simulink model "ElevatorPlant_basic"  (R2015b)
settings: Solver=FixedStepDiscrete  SolverMode=SingleTasking  StartTime=0.0  StopTime=10.0  RelTol=1e-3
(part 2 of 3)

== stateflow chart ElevatorPlant_basic/Elevator Plant ==
  state Init_procedure
    state BLK_Init
      %BLK(LPS0)
      %BLK(LPD1)
      %BLK(LPS1)
      %BLK(LPD2)
      %BLK(LPS2)
      %BLK(LPD3)
    state Replacing
      en:
      SCENDI=true;
    state Closing_all_doors
      state Closing0
        state Timer_close
          state Set_tmr
            en: Q_cl=true;
          state Set
            en:PT_cl=5;
            IN_cl=true;
          state Counting
            en:ET_cl = ET_cl + 1;
            Q_cl=false;
          (junction 9948) -> Init_procedure.Closing_all_doors.Closing0.Timer_close.Set_tmr [order 1] : [ET_cl==PT_cl]
          Init_procedure.Closing_all_doors.Closing0.Timer_close.Set_tmr -> (junction 9949)
          (default) -> Init_procedure.Closing_all_doors.Closing0.Timer_close.Set
          Init_procedure.Closing_all_doors.Closing0.Timer_close.Counting -> (junction 9948)
          (junction 9948) -> (junction 9949) [order 2]
          Init_procedure.Closing_all_doors.Closing0.Timer_close.Set -> (junction 9950)
          (junction 9950) -> Init_procedure.Closing_all_doors.Closing0.Timer_close.Counting [order 1] : [ET_cl<PT_cl]
          (junction 9950) -> (junction 9949) [order 2]
        state BUTT_Temp
          state Butt_temp0
            en: BUT_TEMP = 0;
            FLAG_BT=true;
            LPC0=true;
          state Butt_temp1
            en: BUT_TEMP = 1;
            FLAG_BT=true;
            LPC1=true;
          state Butt_temp2
            en: BUT_TEMP = 2;
            FLAG_BT=true;
            LPC2=true;
          state Butt_temp3
            en: BUT_TEMP = 3;
            FLAG_BT=true;
            LPC3=true;
          (default) -> (junction 13774)
          (junction 13774) -> (junction 13496) [order 1] : [not(FLAG_BT)]
          (junction 13496) -> Init_procedure.Closing_all_doors.Closing0.BUTT_Temp.Butt_temp0 [order 1] : [P0]
          Init_procedure.Closing_all_doors.Closing0.BUTT_Temp.Butt_temp0 -> (junction 13782)
          (junction 13774) -> (junction 13776) [order 2]
          (junction 13496) -> (junction 13769) [order 2]
          (junction 13782) -> (junction 13783)
          (junction 13769) -> Init_procedure.Closing_all_doors.Closing0.BUTT_Temp.Butt_temp1 [order 1] : [P1]
          Init_procedure.Closing_all_doors.Closing0.BUTT_Temp.Butt_temp1 -> (junction 13783)
          (junction 13769) -> (junction 13768) [order 2]
          (junction 13783) -> (junction 13784)
          (junction 13768) -> Init_procedure.Closing_all_doors.Closing0.BUTT_Temp.Butt_temp2 [order 1] : [P2]
          Init_procedure.Closing_all_doors.Closing0.BUTT_Temp.Butt_temp2 -> (junction 13784)
          (junction 13768) -> (junction 13771) [order 2]
          (junction 13784) -> (junction 13785)
          (junction 13771) -> Init_procedure.Closing_all_doors.Closing0.BUTT_Temp.Butt_temp3 [order 1] : [P3]
          Init_procedure.Closing_all_doors.Closing0.BUTT_Temp.Butt_temp3 -> (junction 13785)
          (junction 13771) -> (junction 13779) [order 2]
          (junction 13785) -> (junction 13786)
          (junction 13776) -> (junction 13779)
          (junction 13779) -> (junction 13786)
        state Closing
          en: CP0=Q_cl;
        state Stop_Closing
          en: CP0=false;
          LPS0=false;
          LPS1=false;
          LPD1=false;
          LPS2=false;
          LPD2=false;
          LPD3=false;
          FLAG_OD=false;
          OBS=false;
          ET_cl=0;
          IN_cl=false;
        state Flag_position
          en:FLAG=2;
          FLAG_BT=false;
          BUTTON=BUT_TEMP;
        state Closing1
          en:CP0=true;
        state Flag_floor
          en: FLAG=1;
        state Stop_Closing1
          en:CP0=false;
        Init_procedure.Closing_all_doors.Closing0.Closing -> Init_procedure.Closing_all_doors.Closing0.BUTT_Temp
        (default) -> (junction 9915)
        (junction 9915) -> Init_procedure.Closing_all_doors.Closing0.Timer_close [order 1] : [not(FLAG==0) && not(FLAG==4)]
        Init_procedure.Closing_all_doors.Closing0.Timer_close -> (junction 9914)
        (junction 9914) -> Init_procedure.Closing_all_doors.Closing0.Closing [order 1] : [not(PC0)]
        Init_procedure.Closing_all_doors.Closing0.BUTT_Temp -> (junction 13760)
        (junction 9915) -> (junction 9917) [order 2]
        (junction 9914) -> Init_procedure.Closing_all_doors.Closing0.Stop_Closing [order 2]
        (junction 13760) -> (junction 13757)
        Init_procedure.Closing_all_doors.Closing0.Stop_Closing -> (junction 9916)
        (junction 9916) -> Init_procedure.Closing_all_doors.Closing0.Flag_position [order 1] : [FLAG_BT]
        (junction 9916) -> Init_procedure.Closing_all_doors.Closing0.Flag_floor [order 2]
        Init_procedure.Closing_all_doors.Closing0.Flag_position -> (junction 13754)
        (junction 9917) -> Init_procedure.Closing_all_doors.Closing0.Closing1 [order 1] : [not(PC0)]
        Init_procedure.Closing_all_doors.Closing0.Closing1 -> (junction 13749)
        (junction 9917) -> Init_procedure.Closing_all_doors.Closing0.Stop_Closing1 [order 2]
        (junction 13749) -> (junction 13751)
        Init_procedure.Closing_all_doors.Closing0.Flag_floor -> (junction 13754)
        (junction 13754) -> (junction 13757)
        (junction 13757) -> (junction 13765)
        Init_procedure.Closing_all_doors.Closing0.Stop_Closing1 -> (junction 13751)
        (junction 13751) -> (junction 13765)
      state Closing1
        state BUTT_Temp
          state Butt_temp0
            en: BUT_TEMP = 0;
            FLAG_BT=true;
            LPC0=true;
          state Butt_temp1
            en: BUT_TEMP = 1;
            FLAG_BT=true;
            LPC1=true;
          state Butt_temp2
            en: BUT_TEMP = 2;
            FLAG_BT=true;
            LPC2=true;
          state Butt_temp3
            en: BUT_TEMP = 3;
            FLAG_BT=true;
            LPC3=true;
          (default) -> (junction 14037)
          (junction 14037) -> (junction 14038) [order 1] : [not(FLAG_BT)]
          (junction 14038) -> Init_procedure.Closing_all_doors.Closing1.BUTT_Temp.Butt_temp0 [order 1] : [P0]
          Init_procedure.Closing_all_doors.Closing1.BUTT_Temp.Butt_temp0 -> (junction 14039)
          (junction 14037) -> (junction 14046) [order 2]
          (junction 14038) -> (junction 14041) [order 2]
          (junction 14039) -> (junction 14040)
          (junction 14041) -> Init_procedure.Closing_all_doors.Closing1.BUTT_Temp.Butt_temp1 [order 1] : [P1]
          Init_procedure.Closing_all_doors.Closing1.BUTT_Temp.Butt_temp1 -> (junction 14040)
          (junction 14041) -> (junction 14042) [order 2]
          (junction 14040) -> (junction 14043)
          (junction 14042) -> Init_procedure.Closing_all_doors.Closing1.BUTT_Temp.Butt_temp2 [order 1] : [P2]
          Init_procedure.Closing_all_doors.Closing1.BUTT_Temp.Butt_temp2 -> (junction 14043)
          (junction 14042) -> (junction 14044) [order 2]
          (junction 14043) -> (junction 14045)
          (junction 14044) -> Init_procedure.Closing_all_doors.Closing1.BUTT_Temp.Butt_temp3 [order 1] : [P3]
          Init_procedure.Closing_all_doors.Closing1.BUTT_Temp.Butt_temp3 -> (junction 14045)
          (junction 14044) -> (junction 14047) [order 2]
          (junction 14045) -> (junction 14048)
          (junction 14046) -> (junction 14047)
          (junction 14047) -> (junction 14048)
        state Timer_close
          state Set_tmr
            en: Q_cl=true;
          state Set
            en:PT_cl=5;
            IN_cl=true;
          state Counting
            en:ET_cl = ET_cl + 1;
            Q_cl=false;
          (junction 14022) -> Init_procedure.Closing_all_doors.Closing1.Timer_close.Set_tmr [order 1] : [ET_cl==PT_cl]
          Init_procedure.Closing_all_doors.Closing1.Timer_close.Set_tmr -> (junction 14023)
          (default) -> Init_procedure.Closing_all_doors.Closing1.Timer_close.Set
          Init_procedure.Closing_all_doors.Closing1.Timer_close.Counting -> (junction 14022)
          (junction 14022) -> (junction 14023) [order 2]
          Init_procedure.Closing_all_doors.Closing1.Timer_close.Set -> (junction 14024)
          (junction 14024) -> Init_procedure.Closing_all_doors.Closing1.Timer_close.Counting [order 1] : [ET_cl<PT_cl]
          (junction 14024) -> (junction 14023) [order 2]
        state Closing
          en: CP1=Q_cl;
        state Stop_Closing
          en: CP1=false;
          LPS0=false;
          LPS1=false;
          LPD1=false;
          LPS2=false;
          LPD2=false;
          LPD3=false;
          FLAG_OD=false;
          OBS=false;
          ET_cl=0;
          IN_cl=false;
        state Flag_position
          en:FLAG=2;
          FLAG_BT=false;
          BUTTON=BUT_TEMP;
        state Closing1
          en:CP1=true;
        state Flag_floor
          en: FLAG=1;
        state Stop_Closing1
          en:CP1=false;
        Init_procedure.Closing_all_doors.Closing1.Closing -> Init_procedure.Closing_all_doors.Closing1.BUTT_Temp
        (default) -> (junction 13989)
        (junction 13989) -> Init_procedure.Closing_all_doors.Closing1.Timer_close [order 1] : [not(FLAG==0) && not(FLAG==4)]
        Init_procedure.Closing_all_doors.Closing1.Timer_close -> (junction 13990)
        (junction 13990) -> Init_procedure.Closing_all_doors.Closing1.Closing [order 1] : [not(PC1)]
        Init_procedure.Closing_all_doors.Closing1.BUTT_Temp -> (junction 13991)
        (junction 13989) -> (junction 13993) [order 2]
        (junction 13990) -> Init_procedure.Closing_all_doors.Closing1.Stop_Closing [order 2]
        (junction 13991) -> (junction 13995)
        Init_procedure.Closing_all_doors.Closing1.Stop_Closing -> (junction 13992)
        (junction 13992) -> Init_procedure.Closing_all_doors.Closing1.Flag_position [order 1] : [FLAG_BT]
        (junction 13992) -> Init_procedure.Closing_all_doors.Closing1.Flag_floor [order 2]
        Init_procedure.Closing_all_doors.Closing1.Flag_position -> (junction 13996)
        (junction 13993) -> Init_procedure.Closing_all_doors.Closing1.Closing1 [order 1] : [not(PC1)]
        Init_procedure.Closing_all_doors.Closing1.Closing1 -> (junction 13994)
        (junction 13993) -> Init_procedure.Closing_all_doors.Closing1.Stop_Closing1 [order 2]
        (junction 13994) -> (junction 13997)
        Init_procedure.Closing_all_doors.Closing1.Flag_floor -> (junction 13996)
        (junction 13996) -> (junction 13995)
        (junction 13995) -> (junction 13998)
        Init_procedure.Closing_all_doors.Closing1.Stop_Closing1 -> (junction 13997)
        (junction 13997) -> (junction 13998)
      state Closing2
        state Timer_close
          state Set_tmr
            en: Q_cl=true;
          state Set
            en:PT_cl=5;
            IN_cl=true;
          state Counting
            en:ET_cl = ET_cl + 1;
            Q_cl=false;
          (junction 14114) -> Init_procedure.Closing_all_doors.Closing2.Timer_close.Set_tmr [order 1] : [ET_cl==PT_cl]
          Init_procedure.Closing_all_doors.Closing2.Timer_close.Set_tmr -> (junction 14115)
          (default) -> Init_procedure.Closing_all_doors.Closing2.Timer_close.Set
          Init_procedure.Closing_all_doors.Closing2.Timer_close.Counting -> (junction 14114)
          (junction 14114) -> (junction 14115) [order 2]
          Init_procedure.Closing_all_doors.Closing2.Timer_close.Set -> (junction 14116)
          (junction 14116) -> Init_procedure.Closing_all_doors.Closing2.Timer_close.Counting [order 1] : [ET_cl<PT_cl]
          (junction 14116) -> (junction 14115) [order 2]
        state BUTT_Temp
          state Butt_temp0
            en: BUT_TEMP = 0;
            FLAG_BT=true;
            LPC0=true;
          state Butt_temp1
            en: BUT_TEMP = 1;
            FLAG_BT=true;
            LPC1=true;
          state Butt_temp2
            en: BUT_TEMP = 2;
            FLAG_BT=true;
            LPC2=true;
          state Butt_temp3
            en: BUT_TEMP = 3;
            FLAG_BT=true;
            LPC3=true;
          (default) -> (junction 14129)
          (junction 14129) -> (junction 14130) [order 1] : [not(FLAG_BT)]
          (junction 14130) -> Init_procedure.Closing_all_doors.Closing2.BUTT_Temp.Butt_temp0 [order 1] : [P0]
          Init_procedure.Closing_all_doors.Closing2.BUTT_Temp.Butt_temp0 -> (junction 14131)
          (junction 14129) -> (junction 14138) [order 2]
          (junction 14130) -> (junction 14133) [order 2]
          (junction 14131) -> (junction 14132)
          (junction 14133) -> Init_procedure.Closing_all_doors.Closing2.BUTT_Temp.Butt_temp1 [order 1] : [P1]
          Init_procedure.Closing_all_doors.Closing2.BUTT_Temp.Butt_temp1 -> (junction 14132)
          (junction 14133) -> (junction 14134) [order 2]
          (junction 14132) -> (junction 14135)
          (junction 14134) -> Init_procedure.Closing_all_doors.Closing2.BUTT_Temp.Butt_temp2 [order 1] : [P2]
          Init_procedure.Closing_all_doors.Closing2.BUTT_Temp.Butt_temp2 -> (junction 14135)
          (junction 14134) -> (junction 14136) [order 2]
          (junction 14135) -> (junction 14137)
          (junction 14136) -> Init_procedure.Closing_all_doors.Closing2.BUTT_Temp.Butt_temp3 [order 1] : [P3]
          Init_procedure.Closing_all_doors.Closing2.BUTT_Temp.Butt_temp3 -> (junction 14137)
          (junction 14136) -> (junction 14139) [order 2]
          (junction 14137) -> (junction 14140)
          (junction 14138) -> (junction 14139)
          (junction 14139) -> (junction 14140)
        state Closing
          en: CP2=Q_cl;
        state Stop_Closing
          en: CP2=false;
          LPS0=false;
          LPS1=false;
          LPD1=false;
          LPS2=false;
          LPD2=false;
          LPD3=false;
          FLAG_OD=false;
          OBS=false;
          ET_cl=0;
          IN_cl=false;
        state Flag_position
          en:FLAG=2;
          FLAG_BT=false;
          BUTTON=BUT_TEMP;
        state Closing1
          en:CP2=true;
        state Flag_floor
          en: FLAG=1;
        state Stop_Closing1
          en:CP2=false;
        Init_procedure.Closing_all_doors.Closing2.Closing -> Init_procedure.Closing_all_doors.Closing2.BUTT_Temp
        (default) -> (junction 14081)
        (junction 14081) -> Init_procedure.Closing_all_doors.Closing2.Timer_close [order 1] : [not(FLAG==0) && not(FLAG==4)]
        Init_procedure.Closing_all_doors.Closing2.Timer_close -> (junction 14082)
        (junction 14082) -> Init_procedure.Closing_all_doors.Closing2.Closing [order 1] : [not(PC2)]
        Init_procedure.Closing_all_doors.Closing2.BUTT_Temp -> (junction 14083)
        (junction 14081) -> (junction 14085) [order 2]
        (junction 14082) -> Init_procedure.Closing_all_doors.Closing2.Stop_Closing [order 2]
        (junction 14083) -> (junction 14087)
        Init_procedure.Closing_all_doors.Closing2.Stop_Closing -> (junction 14084)
        (junction 14084) -> Init_procedure.Closing_all_doors.Closing2.Flag_position [order 1] : [FLAG_BT]
        (junction 14084) -> Init_procedure.Closing_all_doors.Closing2.Flag_floor [order 2]
        Init_procedure.Closing_all_doors.Closing2.Flag_position -> (junction 14088)
        (junction 14085) -> Init_procedure.Closing_all_doors.Closing2.Closing1 [order 1] : [not(PC2)]
        Init_procedure.Closing_all_doors.Closing2.Closing1 -> (junction 14086)
        (junction 14085) -> Init_procedure.Closing_all_doors.Closing2.Stop_Closing1 [order 2]
        (junction 14086) -> (junction 14089)
        Init_procedure.Closing_all_doors.Closing2.Flag_floor -> (junction 14088)
        (junction 14088) -> (junction 14087)
        (junction 14087) -> (junction 14090)
        Init_procedure.Closing_all_doors.Closing2.Stop_Closing1 -> (junction 14089)
        (junction 14089) -> (junction 14090)
      state Closing3
        state Timer_close
          state Set_tmr
            en: Q_cl=true;
          state Set
            en:PT_cl=5;
            IN_cl=true;
          state Counting
            en:ET_cl = ET_cl + 1;
            Q_cl=false;
          (junction 14206) -> Init_procedure.Closing_all_doors.Closing3.Timer_close.Set_tmr [order 1] : [ET_cl==PT_cl]
          Init_procedure.Closing_all_doors.Closing3.Timer_close.Set_tmr -> (junction 14207)
          (default) -> Init_procedure.Closing_all_doors.Closing3.Timer_close.Set
          Init_procedure.Closing_all_doors.Closing3.Timer_close.Counting -> (junction 14206)
          (junction 14206) -> (junction 14207) [order 2]
          Init_procedure.Closing_all_doors.Closing3.Timer_close.Set -> (junction 14208)
          (junction 14208) -> Init_procedure.Closing_all_doors.Closing3.Timer_close.Counting [order 1] : [ET_cl<PT_cl]
          (junction 14208) -> (junction 14207) [order 2]
        state BUTT_Temp
          state Butt_temp0
            en: BUT_TEMP = 0;
            FLAG_BT=true;
            LPC0=true;
          state Butt_temp1
            en: BUT_TEMP = 1;
            FLAG_BT=true;
            LPC1=true;
          state Butt_temp2
            en: BUT_TEMP = 2;
            FLAG_BT=true;
            LPC2=true;
          state Butt_temp3
            en: BUT_TEMP = 3;
            FLAG_BT=true;
            LPC3=true;
          (default) -> (junction 14221)
          (junction 14221) -> (junction 14222) [order 1] : [not(FLAG_BT)]
          (junction 14222) -> Init_procedure.Closing_all_doors.Closing3.BUTT_Temp.Butt_temp0 [order 1] : [P0]
          Init_procedure.Closing_all_doors.Closing3.BUTT_Temp.Butt_temp0 -> (junction 14223)
          (junction 14221) -> (junction 14230) [order 2]
          (junction 14222) -> (junction 14225) [order 2]
          (junction 14223) -> (junction 14224)
          (junction 14225) -> Init_procedure.Closing_all_doors.Closing3.BUTT_Temp.Butt_temp1 [order 1] : [P1]
          Init_procedure.Closing_all_doors.Closing3.BUTT_Temp.Butt_temp1 -> (junction 14224)
          (junction 14225) -> (junction 14226) [order 2]
          (junction 14224) -> (junction 14227)
          (junction 14226) -> Init_procedure.Closing_all_doors.Closing3.BUTT_Temp.Butt_temp2 [order 1] : [P2]
          Init_procedure.Closing_all_doors.Closing3.BUTT_Temp.Butt_temp2 -> (junction 14227)
          (junction 14226) -> (junction 14228) [order 2]
          (junction 14227) -> (junction 14229)
          (junction 14228) -> Init_procedure.Closing_all_doors.Closing3.BUTT_Temp.Butt_temp3 [order 1] : [P3]
          Init_procedure.Closing_all_doors.Closing3.BUTT_Temp.Butt_temp3 -> (junction 14229)
          (junction 14228) -> (junction 14231) [order 2]
          (junction 14229) -> (junction 14232)
          (junction 14230) -> (junction 14231)
          (junction 14231) -> (junction 14232)
        state Closing
          en: CP3=Q_cl;
        state Stop_Closing
          en: CP3=false;
          LPS0=false;
          LPS1=false;
          LPD1=false;
          LPS2=false;
          LPD2=false;
          LPD3=false;
          FLAG_OD=false;
          OBS=false;
          ET_cl=0;
          IN_cl=false;
        state Flag_position
          en:FLAG=2;
          FLAG_BT=false;
          BUTTON=BUT_TEMP;
        state Closing1
          en:CP3=true;
        state Flag_floor
          en: FLAG=1;
        state Stop_Closing1
          en:CP3=false;
        Init_procedure.Closing_all_doors.Closing3.Closing -> Init_procedure.Closing_all_doors.Closing3.BUTT_Temp
        (default) -> (junction 14173)
        (junction 14173) -> Init_procedure.Closing_all_doors.Closing3.Timer_close [order 1] : [not(FLAG==0) && not(FLAG==4)]
        Init_procedure.Closing_all_doors.Closing3.Timer_close -> (junction 14174)
        (junction 14174) -> Init_procedure.Closing_all_doors.Closing3.Closing [order 1] : [not(PC3)]
        Init_procedure.Closing_all_doors.Closing3.BUTT_Temp -> (junction 14175)
        (junction 14173) -> (junction 14177) [order 2]
        (junction 14174) -> Init_procedure.Closing_all_doors.Closing3.Stop_Closing [order 2]
        (junction 14175) -> (junction 14179)
        Init_procedure.Closing_all_doors.Closing3.Stop_Closing -> (junction 14176)
        (junction 14176) -> Init_procedure.Closing_all_doors.Closing3.Flag_position [order 1] : [FLAG_BT]
        (junction 14176) -> Init_procedure.Closing_all_doors.Closing3.Flag_floor [order 2]
        Init_procedure.Closing_all_doors.Closing3.Flag_position -> (junction 14180)
        (junction 14177) -> Init_procedure.Closing_all_doors.Closing3.Closing1 [order 1] : [not(PC3)]
        Init_procedure.Closing_all_doors.Closing3.Closing1 -> (junction 14178)
        (junction 14177) -> Init_procedure.Closing_all_doors.Closing3.Stop_Closing1 [order 2]
        (junction 14178) -> (junction 14181)
        Init_procedure.Closing_all_doors.Closing3.Flag_floor -> (junction 14180)
        (junction 14180) -> (junction 14179)
        (junction 14179) -> (junction 14182)
        Init_procedure.Closing_all_doors.Closing3.Stop_Closing1 -> (junction 14181)
        (junction 14181) -> (junction 14182)
      (default) -> Init_procedure.Closing_all_doors.Closing0
      Init_procedure.Closing_all_doors.Closing1 -> Init_procedure.Closing_all_doors.Closing2
      Init_procedure.Closing_all_doors.Closing0 -> Init_procedure.Closing_all_doors.Closing1
      Init_procedure.Closing_all_doors.Closing2 -> Init_procedure.Closing_all_doors.Closing3
    state Replaced
      en:
      SCENDI=false;
    state End_init
      en:
      LPS0=false;LPS1=false;
      LPS2=false;LPD2=false;
      LPD3=false;LPD1=false;
      FLAG=1;
    Init_procedure.Replacing -> (junction 13744)
    BLK_Init -> Closing_all_doors
    Closing_all_doors -> (junction 4531)
    (junction 4531) -> Init_procedure.Replacing [order 1] : [not(RPC0) && not(RPC1) && not(RPC2) && not(RPC3)]
    (default) -> BLK_Init
    (junction 13744) -> (junction 13732)
    (junction 4531) -> Init_procedure.Replaced [order 2]
    Init_procedure.Replaced -> (junction 13732)
    (junction 13732) -> (junction 13735)
    (junction 13735) -> (junction 13739) [order 2]
    (junction 13735) -> End_init [order 1] : [(RPC0 ||RPC1 ||RPC2 ||RPC3) && (PC0 && PC1 && PC2 && PC3)]
    (junction 13739) -> (junction 13741)
    End_init -> (junction 13737)
    (junction 13737) -> (junction 13741)
  state Blackout
    state OFF
      en:	FLAG_BO=true;
      AP0=false;
      AP1=false;
      AP2=false;
      AP3=false;
      CP0=false;
      CP1=false;
      CP2=false;
      CP3=false;
      SALI=false;
      SCENDI=false;
      LL=false;
      LPC0=false;
      LPC1=false;
      LPC2=false;
      LPC3=false;
      LPS0=false;
      LPS1=false;
      LPD1=false;
      LPS2=false;
      LPD2=false;
      LPD3=false;
      FLAG=5;
      IN_LL=false; ET_LL=0;
    state Start_recovery
      en:
      FLAG_REC=true;
      FLAG=4;
    state ON
      en:
      LL=true;
    state Recovery_finished
    OFF -> (junction 13581)
    (default) -> (junction 4492)
    (junction 4492) -> OFF [order 1] : [BO && not(FLAG_BO) && not(RECOVERY)]
    (junction 4492) -> (junction 13599) [order 2]
    (junction 13581) -> Start_recovery [order 1] : [RECOVERY]
    Start_recovery -> (junction 13584)
    (junction 13599) -> ON [order 1] : [not(BO) && not(RECOVERY)]
    ON -> (junction 13581)
    (junction 13581) -> Recovery_finished [order 2]
    Recovery_finished -> (junction 13584)
    (junction 13599) -> (junction 13728) [order 2]
    (junction 13726) -> (junction 13581)
    (junction 13728) -> (junction 13726)
  state Fire_detection
    state Firing
      en:FLAG=4;
      FLAG_EMG=true;
      SALI=false;
    state NOT_fire
    (default) -> (junction 13568)
    (junction 13568) -> Firing [order 1] : [FIRE]
    Firing -> (junction 13579)
    (junction 13568) -> NOT_fire [order 2]
    NOT_fire -> (junction 13579)
  state Floor_detection
    state F0
      en:
      FLOOR=0;
      LPC0=true;
    state No_floor
    state NOT_F0
      en:
      LPC0=false;
    state F1
      en:
      FLOOR=1;
      LPC1=true;
    state NOT_F1
      en:
      LPC1=false;
    state F2
      en:
      FLOOR=2;
      LPC2=true;
    state NOT_F2
      en:
      LPC2=false;
    state F3
      en:
      FLOOR=3;
      LPC3=true;
    state F4
      en:
      LPC3=false;
    (junction 4501) -> F0 [order 1] : [RPC0]
    Floor_detection.No_floor -> (junction 4501)
    F0 -> (junction 13681)
    (default) -> Floor_detection.No_floor
    (junction 4501) -> (junction 13667) [order 2]
    (junction 13667) -> NOT_F0 [order 1] : [not(BUT_TEMP==0)]
    NOT_F0 -> (junction 13681)
    (junction 13667) -> (junction 13684) [order 2]
    (junction 13681) -> (junction 13707)
    (junction 13707) -> (junction 13684)
    (junction 13684) -> (junction 4502)
    (junction 4502) -> F1 [order 1] : [RPC1]
    (junction 4502) -> (junction 13669) [order 2]
    F1 -> (junction 13688)
    (junction 13669) -> NOT_F1 [order 1] : [not(BUT_TEMP==1)]
    (junction 13669) -> (junction 13691) [order 2]
    NOT_F1 -> (junction 13688)
    (junction 13688) -> (junction 13705)
    (junction 13705) -> (junction 13691)
    (junction 13691) -> (junction 4503)
    (junction 4503) -> F2 [order 1] : [RPC2]
    F2 -> (junction 13709)
    (junction 4503) -> (junction 13671) [order 2]
    (junction 13671) -> NOT_F2 [order 1] : [not(BUT_TEMP==2)]
    NOT_F2 -> (junction 13709)
    (junction 13671) -> (junction 13695) [order 2]
    (junction 13709) -> (junction 13702)
    (junction 13702) -> (junction 13695)
    (junction 13695) -> (junction 4504)
    F3 -> (junction 13710)
    (junction 4504) -> F3 [order 1] : [RPC3]
    (junction 4504) -> (junction 13673) [order 2]
    (junction 13673) -> F4 [order 1] : [not(BUT_TEMP==3)]
    F4 -> (junction 13710)
    (junction 13673) -> (junction 13715) [order 2]
    (junction 13710) -> (junction 13713)
    (junction 13715) -> (junction 13713)
  state Button_detection
    state BUTTON_0
      en:
      BUTTON=0;
      FLAG=2;
      IN_LL=false; ET_LL=0;
    state No_button
    state Supply_OFF
      en:
      LL=not(Q_LL);
    state Timer_LL
      state Set_tmr
        en:
        Q_LL=true;
      state Counting
        en:
        ET_LL = ET_LL + 1;
        Q_LL=false;
      state Set
        en:
        IN_LL=true;
        PT_LL=10;
      (junction 4546) -> Button_detection.Timer_LL.Set_tmr [order 1] : [ET_LL==PT_LL]
      Button_detection.Timer_LL.Set_tmr -> (junction 4547)
      Button_detection.Timer_LL.Counting -> (junction 4546)
      (junction 4546) -> (junction 4547) [order 2]
      (default) -> Button_detection.Timer_LL.Set
      Button_detection.Timer_LL.Set -> (junction 4545)
      (junction 4545) -> Button_detection.Timer_LL.Counting [order 1] : [ET_LL<PT_LL]
      (junction 4545) -> (junction 4547) [order 2]
    state BUTTON_1
      en:
      BUTTON=1;
      FLAG=2;
      IN_LL=false; ET_LL=0;
    state BUTTON_2
      en:
      BUTTON=2;
      FLAG=2;
      IN_LL=false; ET_LL=0;
    state BUTTON_3
      en:
      BUTTON=3;
      FLAG=2;
      IN_LL=false; ET_LL=0;
    state STOP
      en:
      IN_LL=false; ET_LL=0;
      FLAG=1;
    state Timer_EME
      state Set_tmr
        en:
        Q_EME=true;
      state Counting
        en:
        ET_EME= ET_EME + 1;
        Q_EME=false;
      state Set
        en:
        IN_EME=true;
        PT_EME=3;
      (junction 4593) -> Button_detection.Timer_EME.Set_tmr [order 1] : [ET_EME==PT_EME]
      Button_detection.Timer_EME.Set_tmr -> (junction 4594)
      Button_detection.Timer_EME.Counting -> (junction 4593)
      (junction 4593) -> (junction 4594) [order 2]
      (default) -> Button_detection.Timer_EME.Set
      Button_detection.Timer_EME.Set -> (junction 4595)
      (junction 4595) -> Button_detection.Timer_EME.Counting [order 1] : [ET_EME<PT_EME]
      (junction 4595) -> (junction 4594) [order 2]
    state EME
      en:
      FLAG_EME=true;
      FLAG=4;
    state Remain_here
      en:
      FLAG=1;
    state NOT_STOP
      en:
      IN_EME=false;
      ET_EME=0;
    (default) -> No_button
    (junction 14266) -> Timer_LL [order 1] : [FLAG_STOP]
    Supply_OFF -> (junction 4167)
    (junction 4167) -> BUTTON_0 [order 1] : [P0|| PS0]
    BUTTON_0 -> (junction 14276)
    No_button -> (junction 14266)
    Timer_LL -> Supply_OFF
    (junction 14266) -> (junction 14295) [order 2]
    (junction 4167) -> (junction 14268) [order 2]
    (junction 14276) -> (junction 14277)
    (junction 14268) -> BUTTON_1 [order 1] : [P1|| PS1|| PD1]
    BUTTON_1 -> (junction 14277)
    (junction 14268) -> (junction 14270) [order 2]
    (junction 14277) -> (junction 14278)
    (junction 14270) -> BUTTON_2 [order 1] : [P2 || PS2 || PD2]
    BUTTON_2 -> (junction 14278)
    (junction 14270) -> (junction 14272) [order 2]
    (junction 14278) -> (junction 14279)
    (junction 25236) -> (junction 14291) [order 2]
    (junction 14272) -> BUTTON_3 [order 1] : [P3 || PD3]
    BUTTON_3 -> (junction 14279)
    (junction 14272) -> Remain_here [order 2]
    (junction 14279) -> (junction 14289)
    (junction 4567) -> STOP [order 1] : [STOP]
    STOP -> Timer_EME
    Timer_EME -> (junction 25236)
    (junction 25236) -> EME [order 1] : [Q_EME]
    EME -> (junction 14291)
    NOT_STOP -> (junction 14291)
    (junction 14291) -> (junction 14297)
    Remain_here -> (junction 14289)
    (junction 14289) -> (junction 4567) : {BUT_TEMP=BUTTON}
    (junction 4567) -> NOT_STOP [order 2]
    (junction 14295) -> (junction 14297)
  state Position_control
    state BUSY
      en:LPS0=true;
      LPS1=true;
      LPD1=true;
      LPS2=true;
      LPD2=true;
      LPD3=true;
    state MOVING_UP
      en:SALI=true;
      MOTION=0;
      FLAG_STOP=false;
      %BLK_TARGET()
    state MOVING_DOWN
      en:SCENDI=true;
      MOTION=1;
      FLAG_STOP=false;
      %BLK_TARGET()
    state AFTER_STOP
      state DOWN_STOP
        en: SCENDI=true;
        %BLK_TARGET();
      state NOT_DOWN
        en: FLAG_STOP=false;
      state UP_STOP
        en: SALI=true;
        %BLK_TARGET();
      state NOT_UP
        en: FLAG_STOP=false;
      (default) -> (junction 8506)
      (junction 8506) -> (junction 8505) [order 1] : [MOTION==0]
      (junction 8505) -> DOWN_STOP [order 1] : [not(( RPC0==true && BUTTON==0)||( RPC1==true && BUTTON==1)||( RPC2==true && BUTTON==2)||( RPC3==true && BUTTON==3)||(STOP==true))]
      (junction 8506) -> (junction 8507) [order 2] : [MOTION==1]
      (junction 8505) -> NOT_DOWN [order 2]
      DOWN_STOP -> (junction 14323)
      NOT_DOWN -> (junction 14323)
      (junction 14323) -> (junction 14326)
      (junction 8507) -> UP_STOP [order 1] : [not(( RPC0==true && BUTTON==0)||( RPC1==true && BUTTON==1)||( RPC2==true && BUTTON==2)||( RPC3==true && BUTTON==3)||(STOP==true))]
      (junction 8507) -> NOT_UP [order 2]
      UP_STOP -> (junction 14320)
      NOT_UP -> (junction 14320)
      (junction 14320) -> (junction 14326)
    state FINISH_POSITIONING
      en:FLAG=3;
    state STOP_CONDITION
      en:FLAG=1;
      FLAG_STOP=true;
    (default) -> BUSY
    BUSY -> (junction 8494)
    (junction 8494) -> MOVING_UP [order 1] : [BUTTON>FLOOR && not(STOP)]
    MOVING_UP -> (junction 14309)
    (junction 8494) -> (junction 14302) [order 2]
    (junction 14309) -> (junction 14310)
    (junction 14302) -> MOVING_DOWN [order 1] : [BUTTON<FLOOR && not(STOP)]
    MOVING_DOWN -> (junction 14310)
    (junction 14302) -> (junction 14305) [order 2]
    (junction 14310) -> (junction 14311)
    (junction 14305) -> AFTER_STOP [order 1] : [BUTTON==FLOOR && FLAG_STOP]
    AFTER_STOP -> (junction 14311)
    (junction 14305) -> (junction 25225) [order 2] : {SALI=false;
        | SCENDI=false;
        | LPC0=false;
        | LPC1=false;
        | LPC2=false;
        | LPC3=false;}
    (junction 14311) -> (junction 14317)
    (junction 25225) -> FINISH_POSITIONING [order 1] : [RPC0==true ||RPC1==true ||RPC2==true ||RPC3==true]
    (junction 25225) -> STOP_CONDITION [order 2]
    FINISH_POSITIONING -> (junction 25226)
    (junction 25226) -> (junction 14317)
    STOP_CONDITION -> (junction 25226)
  state OpCl_doors
    state OpCl_0
      state Closing0
        state Timer_close
          state Set_tmr
            en: Q_cl=true;
          state Set
            en:PT_cl=5;
            IN_cl=true;
          state Counting
            en:ET_cl = ET_cl + 1;
            Q_cl=false;
          (junction 14764) -> OpCl_doors.OpCl_0.Closing0.Timer_close.Set_tmr [order 1] : [ET_cl==PT_cl]
          OpCl_doors.OpCl_0.Closing0.Timer_close.Set_tmr -> (junction 14765)
          (default) -> OpCl_doors.OpCl_0.Closing0.Timer_close.Set
          OpCl_doors.OpCl_0.Closing0.Timer_close.Counting -> (junction 14764)
          (junction 14764) -> (junction 14765) [order 2]
          OpCl_doors.OpCl_0.Closing0.Timer_close.Set -> (junction 14766)
          (junction 14766) -> OpCl_doors.OpCl_0.Closing0.Timer_close.Counting [order 1] : [ET_cl<PT_cl]
          (junction 14766) -> (junction 14765) [order 2]
        state BUTT_Temp
          state Butt_temp0
            en: BUT_TEMP = 0;
            FLAG_BT=true;
            LPC0=true;
          state Butt_temp1
            en: BUT_TEMP = 1;
            FLAG_BT=true;
            LPC1=true;
          state Butt_temp2
            en: BUT_TEMP = 2;
            FLAG_BT=true;
            LPC2=true;
          state Butt_temp3
            en: BUT_TEMP = 3;
            FLAG_BT=true;
            LPC3=true;
          (default) -> (junction 14779)
          (junction 14779) -> (junction 14780) [order 1] : [not(FLAG_BT)]
          (junction 14780) -> OpCl_doors.OpCl_0.Closing0.BUTT_Temp.Butt_temp0 [order 1] : [P0]
          OpCl_doors.OpCl_0.Closing0.BUTT_Temp.Butt_temp0 -> (junction 14781)
          (junction 14779) -> (junction 14788) [order 2]
          (junction 14780) -> (junction 14783) [order 2]
          (junction 14781) -> (junction 14782)
          (junction 14783) -> OpCl_doors.OpCl_0.Closing0.BUTT_Temp.Butt_temp1 [order 1] : [P1]
          OpCl_doors.OpCl_0.Closing0.BUTT_Temp.Butt_temp1 -> (junction 14782)
          (junction 14783) -> (junction 14784) [order 2]
          (junction 14782) -> (junction 14785)
          (junction 14784) -> OpCl_doors.OpCl_0.Closing0.BUTT_Temp.Butt_temp2 [order 1] : [P2]
          OpCl_doors.OpCl_0.Closing0.BUTT_Temp.Butt_temp2 -> (junction 14785)
          (junction 14784) -> (junction 14786) [order 2]
          (junction 14785) -> (junction 14787)
          (junction 14786) -> OpCl_doors.OpCl_0.Closing0.BUTT_Temp.Butt_temp3 [order 1] : [P3]
          OpCl_doors.OpCl_0.Closing0.BUTT_Temp.Butt_temp3 -> (junction 14787)
          (junction 14786) -> (junction 14789) [order 2]
          (junction 14787) -> (junction 14790)
          (junction 14788) -> (junction 14789)
          (junction 14789) -> (junction 14790)
        state Closing
          en: CP0=Q_cl;
        state Stop_Closing
          en: CP0=false;
          LPS0=false;
          LPS1=false;
          LPD1=false;
          LPS2=false;
          LPD2=false;
          LPD3=false;
          FLAG_OD=false;
          OBS=false;
          ET_cl=0;
          IN_cl=false;
        state Flag_position
          en:FLAG=2;
          FLAG_BT=false;
          BUTTON=BUT_TEMP;
        state Closing1
          en:CP0=true;
        state Flag_floor
          en: FLAG=1;
        state Stop_Closing1
          en:CP0=false;
        OpCl_doors.OpCl_0.Closing0.Closing -> OpCl_doors.OpCl_0.Closing0.BUTT_Temp
        (default) -> (junction 14731)
        (junction 14731) -> OpCl_doors.OpCl_0.Closing0.Timer_close [order 1] : [not(FLAG==0) && not(FLAG==4)]
        OpCl_doors.OpCl_0.Closing0.Timer_close -> (junction 14732)
        (junction 14732) -> OpCl_doors.OpCl_0.Closing0.Closing [order 1] : [not(PC0)]
        OpCl_doors.OpCl_0.Closing0.BUTT_Temp -> (junction 14733)
        (junction 14731) -> (junction 14735) [order 2]
        (junction 14732) -> OpCl_doors.OpCl_0.Closing0.Stop_Closing [order 2]
        (junction 14733) -> (junction 14737)
        OpCl_doors.OpCl_0.Closing0.Stop_Closing -> (junction 14734)
        (junction 14734) -> OpCl_doors.OpCl_0.Closing0.Flag_position [order 1] : [FLAG_BT]
        (junction 14734) -> OpCl_doors.OpCl_0.Closing0.Flag_floor [order 2]
        OpCl_doors.OpCl_0.Closing0.Flag_position -> (junction 14738)
        (junction 14735) -> OpCl_doors.OpCl_0.Closing0.Closing1 [order 1] : [not(PC0)]
        OpCl_doors.OpCl_0.Closing0.Closing1 -> (junction 14736)
        (junction 14735) -> OpCl_doors.OpCl_0.Closing0.Stop_Closing1 [order 2]
        (junction 14736) -> (junction 14739)
        OpCl_doors.OpCl_0.Closing0.Flag_floor -> (junction 14738)
        (junction 14738) -> (junction 14737)
        (junction 14737) -> (junction 14740)
        OpCl_doors.OpCl_0.Closing0.Stop_Closing1 -> (junction 14739)
        (junction 14739) -> (junction 14740)
      state StopClosing
        en: CP0=false;
        FLAG_OD=false;
      state Opening0
        state Opening
          en:AP0=Q_op;
        state Stop_Opening
          en:AP0=false;
          FLAG_OD=true;
          OBS=true;
          IN_op=false;
          ET_op=0;
        state Timer_open
          state Set_tmr
            en: Q_op=true;
          state Set
            en:PT_op=2;
            IN_op=true;
          state Counting
            en:ET_op = ET_op + 1;
            Q_op=false;
          (junction 15302) -> OpCl_doors.OpCl_0.Opening0.Timer_open.Set_tmr [order 1] : [ET_op==PT_op]
          OpCl_doors.OpCl_0.Opening0.Timer_open.Set_tmr -> (junction 15303)
          (default) -> OpCl_doors.OpCl_0.Opening0.Timer_open.Set
          OpCl_doors.OpCl_0.Opening0.Timer_open.Counting -> (junction 15302)
          (junction 15302) -> (junction 15303) [order 2]
          OpCl_doors.OpCl_0.Opening0.Timer_open.Set -> (junction 15304)
          (junction 15304) -> OpCl_doors.OpCl_0.Opening0.Timer_open.Counting [order 1] : [ET_op<PT_op]
          (junction 15304) -> (junction 15303) [order 2]
        state BUTT_Temp
          state Butt_temp0
            en: BUT_TEMP = 0;
            FLAG_BT=true;
            LPC0=true;
          state Butt_temp1
            en: BUT_TEMP = 1;
            FLAG_BT=true;
            LPC1=true;
          state Butt_temp2
            en: BUT_TEMP = 2;
            FLAG_BT=true;
            LPC2=true;
          state Butt_temp3
            en: BUT_TEMP = 3;
            FLAG_BT=true;
            LPC3=true;
          (default) -> (junction 20090)
          (junction 20090) -> (junction 20091) [order 1] : [not(FLAG_BT)]
          (junction 20091) -> OpCl_doors.OpCl_0.Opening0.BUTT_Temp.Butt_temp0 [order 1] : [P0]
          OpCl_doors.OpCl_0.Opening0.BUTT_Temp.Butt_temp0 -> (junction 20092)
          (junction 20091) -> (junction 20094) [order 2]
          (junction 20092) -> (junction 20093)
          (junction 20090) -> (junction 20101) [order 2]
          OpCl_doors.OpCl_0.Opening0.BUTT_Temp.Butt_temp1 -> (junction 20093)
          (junction 20094) -> OpCl_doors.OpCl_0.Opening0.BUTT_Temp.Butt_temp1 [order 1] : [P1]
          (junction 20093) -> (junction 20096)
          (junction 20094) -> (junction 20095) [order 2]
          (junction 20095) -> OpCl_doors.OpCl_0.Opening0.BUTT_Temp.Butt_temp2 [order 1] : [P2]
          OpCl_doors.OpCl_0.Opening0.BUTT_Temp.Butt_temp2 -> (junction 20096)
          (junction 20095) -> (junction 20097) [order 2]
          (junction 20096) -> (junction 20098)
          (junction 20097) -> OpCl_doors.OpCl_0.Opening0.BUTT_Temp.Butt_temp3 [order 1] : [P3]
          OpCl_doors.OpCl_0.Opening0.BUTT_Temp.Butt_temp3 -> (junction 20098)
          (junction 20098) -> (junction 20100)
          (junction 20097) -> (junction 20099) [order 2]
          (junction 20100) -> (junction 20099)
          (junction 20099) -> (junction 20102)
          (junction 20101) -> (junction 20102)
        state People_IN
          state Check_People_IN
            en:
            COUNTER_IN=false;
          state Ready_IN
            en:
            IN_DEL_IN=false;
            ET_DEL_IN=0;
          state People_KID_IN
            en:
            WEIGHT=WEIGHT+30;
            KIDS=KIDS+1;
          state DELAY_IN
            state Set_tmr
              en:
              Q_DEL_IN=true;
            state Counting
              en:
              ET_DEL_IN = ET_DEL_IN + 1;
              Q_DEL_IN=false;
            state Set
              en:
              IN_DEL_IN=true;
              PT_DEL_IN=0.05;
            (junction 15383) -> OpCl_doors.OpCl_0.Opening0.People_IN.DELAY_IN.Set_tmr [order 1] : [ET_DEL_IN==PT_DEL_IN]
            OpCl_doors.OpCl_0.Opening0.People_IN.DELAY_IN.Set_tmr -> (junction 15384)
            OpCl_doors.OpCl_0.Opening0.People_IN.DELAY_IN.Counting -> (junction 15383)
            (junction 15383) -> (junction 15384) [order 2]
            (default) -> OpCl_doors.OpCl_0.Opening0.People_IN.DELAY_IN.Set
            OpCl_doors.OpCl_0.Opening0.People_IN.DELAY_IN.Set -> (junction 15385)
            (junction 15385) -> OpCl_doors.OpCl_0.Opening0.People_IN.DELAY_IN.Counting [order 1] : [ET_DEL_IN<PT_DEL_IN]
            (junction 15385) -> (junction 15384) [order 2]
          state People_WOMAN_IN
            en:
            WEIGHT=WEIGHT+55;
            WOMEN=WOMEN+1;
          state People_MAN_IN
            en:
            WEIGHT=WEIGHT+75;
            MEN=MEN+1;
          state People_FATGUY_IN
            en:
            WEIGHT=WEIGHT+100;
            FATGUYS=FATGUYS+1;
          state Re_Ready_IN
            en:
            COUNTER_IN=true;
          OpCl_doors.OpCl_0.Opening0.People_IN.Check_People_IN -> (junction 15328)
          (junction 15328) -> OpCl_doors.OpCl_0.Opening0.People_IN.People_KID_IN [order 1] : [KID_IN]
          OpCl_doors.OpCl_0.Opening0.People_IN.People_KID_IN -> (junction 15329)
          OpCl_doors.OpCl_0.Opening0.People_IN.DELAY_IN -> (junction 15330)
          (junction 15330) -> OpCl_doors.OpCl_0.Opening0.People_IN.Ready_IN [order 1] : [Q_DEL_IN]
          (default) -> OpCl_doors.OpCl_0.Opening0.People_IN.DELAY_IN
          OpCl_doors.OpCl_0.Opening0.People_IN.Ready_IN -> (junction 15331)
          (junction 15331) -> OpCl_doors.OpCl_0.Opening0.People_IN.Check_People_IN [order 1] : [COUNTER_IN]
          (junction 15328) -> (junction 15333) [order 2]
          (junction 15329) -> (junction 15332)
          (junction 15330) -> (junction 15342) [order 2]
          (junction 15331) -> (junction 15341) [order 2]
          (junction 15333) -> OpCl_doors.OpCl_0.Opening0.People_IN.People_WOMAN_IN [order 1] : [WOMAN_IN]
          OpCl_doors.OpCl_0.Opening0.People_IN.People_WOMAN_IN -> (junction 15332)
          (junction 15333) -> (junction 15334) [order 2]
          (junction 15332) -> (junction 15335)
          (junction 15334) -> OpCl_doors.OpCl_0.Opening0.People_IN.People_MAN_IN [order 1] : [MAN_IN]
          OpCl_doors.OpCl_0.Opening0.People_IN.People_MAN_IN -> (junction 15335)
          (junction 15334) -> (junction 15336) [order 2]
          (junction 15335) -> (junction 15337)
          (junction 15336) -> OpCl_doors.OpCl_0.Opening0.People_IN.People_FATGUY_IN [order 1] : [FATGUY_IN]
          OpCl_doors.OpCl_0.Opening0.People_IN.People_FATGUY_IN -> (junction 15337)
          (junction 15336) -> (junction 15338) [order 2]
          (junction 15337) -> (junction 15339)
          (junction 15338) -> (junction 15339)
          (junction 15339) -> (junction 15340)
          (junction 15341) -> (junction 15340)
          (junction 15340) -> (junction 15343)
          (junction 15342) -> (junction 15343)
          (junction 15343) -> (junction 15344)
          (junction 15344) -> OpCl_doors.OpCl_0.Opening0.People_IN.Re_Ready_IN [order 1] : [not(KID_IN|| WOMAN_IN || MAN_IN || FATGUY_IN)]
          (junction 15344) -> (junction 15345) [order 2]
          OpCl_doors.OpCl_0.Opening0.People_IN.Re_Ready_IN -> (junction 15345)
        state People_OUT
          state Ready_OUT
            en:
            IN_DEL_OUT=false;
            ET_DEL_OUT=0;
          state Check_People_OUT
            en:
            COUNTER_OUT=false;
          state People_KID_OUT
            en:
            WEIGHT=WEIGHT-30;
            KIDS=KIDS-1;
          state DELAY_OUT
            state Set_tmr
              en:
              Q_DEL_OUT=true;
            state Counting
              en:
              ET_DEL_OUT = ET_DEL_OUT + 1;
              Q_DEL_OUT=false;
            state Set
              en:
              IN_DEL_OUT=true;
              PT_DEL_OUT=0.05;
            (junction 15457) -> OpCl_doors.OpCl_0.Opening0.People_OUT.DELAY_OUT.Set_tmr [order 1] : [ET_DEL_OUT==PT_DEL_OUT]
            OpCl_doors.OpCl_0.Opening0.People_OUT.DELAY_OUT.Set_tmr -> (junction 15458)
            OpCl_doors.OpCl_0.Opening0.People_OUT.DELAY_OUT.Counting -> (junction 15457)
            (junction 15457) -> (junction 15458) [order 2]
            (default) -> OpCl_doors.OpCl_0.Opening0.People_OUT.DELAY_OUT.Set
            OpCl_doors.OpCl_0.Opening0.People_OUT.DELAY_OUT.Set -> (junction 15459)
            (junction 15459) -> OpCl_doors.OpCl_0.Opening0.People_OUT.DELAY_OUT.Counting [order 1] : [ET_DEL_OUT<PT_DEL_OUT]
            (junction 15459) -> (junction 15458) [order 2]
          state People_WOMAN_OUT
            en:
            WEIGHT=WEIGHT-55;
            WOMEN=WOMEN-1;
          state People_MAN_OUT
            en:
            WEIGHT=WEIGHT-75;
            MEN=MEN-1;
          state People_FATGUY_OUT
            en:
            WEIGHT=WEIGHT-100;
            FATGUYS=FATGUYS-1;
          state Re_Ready_OUT
            en:
            COUNTER_OUT=true;
          (default) -> OpCl_doors.OpCl_0.Opening0.People_OUT.DELAY_OUT
          OpCl_doors.OpCl_0.Opening0.People_OUT.DELAY_OUT -> (junction 15402)
          (junction 15402) -> OpCl_doors.OpCl_0.Opening0.People_OUT.Ready_OUT [order 1] : [Q_DEL_OUT]
          OpCl_doors.OpCl_0.Opening0.People_OUT.Ready_OUT -> (junction 15403)
          (junction 15403) -> OpCl_doors.OpCl_0.Opening0.People_OUT.Check_People_OUT [order 1] : [COUNTER_OUT]
          OpCl_doors.OpCl_0.Opening0.People_OUT.Check_People_OUT -> (junction 15404)
          (junction 15404) -> OpCl_doors.OpCl_0.Opening0.People_OUT.People_KID_OUT [order 1] : [KID_OUT && KIDS>0 ]
          OpCl_doors.OpCl_0.Opening0.People_OUT.People_KID_OUT -> (junction 15405)
          (junction 15402) -> (junction 15416) [order 2]
          (junction 15403) -> (junction 15414) [order 2]
          (junction 15404) -> (junction 15406) [order 2]
          (junction 15405) -> (junction 15407)
          (junction 15406) -> OpCl_doors.OpCl_0.Opening0.People_OUT.People_WOMAN_OUT [order 1] : [WOMAN_OUT && WOMEN>0]
          OpCl_doors.OpCl_0.Opening0.People_OUT.People_WOMAN_OUT -> (junction 15407)
          (junction 15406) -> (junction 15409) [order 2]
          (junction 15407) -> (junction 15408)
          (junction 15409) -> OpCl_doors.OpCl_0.Opening0.People_OUT.People_MAN_OUT [order 1] : [MAN_OUT && MEN>0]
          OpCl_doors.OpCl_0.Opening0.People_OUT.People_MAN_OUT -> (junction 15408)
          (junction 15409) -> (junction 15410) [order 2]
          (junction 15408) -> (junction 15411)
          (junction 15410) -> OpCl_doors.OpCl_0.Opening0.People_OUT.People_FATGUY_OUT [order 1] : [FATGUY_OUT && FATGUYS>0]
          OpCl_doors.OpCl_0.Opening0.People_OUT.People_FATGUY_OUT -> (junction 15411)
          (junction 15410) -> (junction 15413) [order 2]
          (junction 15411) -> (junction 15412)
          (junction 15413) -> (junction 15412)
          (junction 15412) -> (junction 15415)
          (junction 15414) -> (junction 15415)
          (junction 15415) -> (junction 15417)
          (junction 15416) -> (junction 15417)
          (junction 15417) -> (junction 15418)
          (junction 15418) -> OpCl_doors.OpCl_0.Opening0.People_OUT.Re_Ready_OUT [order 1] : [not(KID_OUT || WOMAN_OUT || MAN_OUT || FATGUY_OUT)]
          (junction 15418) -> (junction 15419) [order 2]
          OpCl_doors.OpCl_0.Opening0.People_OUT.Re_Ready_OUT -> (junction 15419)
        state BUTT_Temp1
          state Butt_temp0
            en: BUT_TEMP = 0;
            FLAG_BT=true;
            LPC0=true;
          state Butt_temp1
            en: BUT_TEMP = 1;
            FLAG_BT=true;
            LPC1=true;
          state Butt_temp2
            en: BUT_TEMP = 2;
            FLAG_BT=true;
            LPC2=true;
          state Butt_temp3
            en: BUT_TEMP = 3;
            FLAG_BT=true;
            LPC3=true;
          (default) -> (junction 20130)
          (junction 20130) -> (junction 20131) [order 1] : [not(FLAG_BT)]
          (junction 20131) -> OpCl_doors.OpCl_0.Opening0.BUTT_Temp1.Butt_temp0 [order 1] : [P0]
          OpCl_doors.OpCl_0.Opening0.BUTT_Temp1.Butt_temp0 -> (junction 20132)
          (junction 20131) -> (junction 20134) [order 2]
          (junction 20132) -> (junction 20133)
          (junction 20130) -> (junction 20141) [order 2]
          OpCl_doors.OpCl_0.Opening0.BUTT_Temp1.Butt_temp1 -> (junction 20133)
          (junction 20134) -> OpCl_doors.OpCl_0.Opening0.BUTT_Temp1.Butt_temp1 [order 1] : [P1]
          (junction 20133) -> (junction 20136)
          (junction 20134) -> (junction 20135) [order 2]
          (junction 20135) -> OpCl_doors.OpCl_0.Opening0.BUTT_Temp1.Butt_temp2 [order 1] : [P2]
          OpCl_doors.OpCl_0.Opening0.BUTT_Temp1.Butt_temp2 -> (junction 20136)
          (junction 20135) -> (junction 20137) [order 2]
          (junction 20136) -> (junction 20138)
          (junction 20137) -> OpCl_doors.OpCl_0.Opening0.BUTT_Temp1.Butt_temp3 [order 1] : [P3]
          OpCl_doors.OpCl_0.Opening0.BUTT_Temp1.Butt_temp3 -> (junction 20138)
          (junction 20138) -> (junction 20140)
          (junction 20137) -> (junction 20139) [order 2]
          (junction 20140) -> (junction 20139)
          (junction 20139) -> (junction 20142)
          (junction 20141) -> (junction 20142)
        state Opening1
          en:AP0=true;
        state Stop_Opening1
          en: AP0=false;
          FLAG_OD=true;
          IN_cl=false;
          ET_cl=0;
        (junction 15269) -> (junction 15268)
        OpCl_doors.OpCl_0.Opening0.Opening -> (junction 15269)
        OpCl_doors.OpCl_0.Opening0.Stop_Opening -> (junction 15269)
        (junction 15268) -> (junction 15274)
        (junction 15270) -> OpCl_doors.OpCl_0.Opening0.Opening [order 1] : [not(PA0)]
        OpCl_doors.OpCl_0.Opening0.Timer_open -> (junction 20169)
        (junction 20169) -> OpCl_doors.OpCl_0.Opening0.BUTT_Temp [order 1] : [not(FLAG==4)]
        OpCl_doors.OpCl_0.Opening0.BUTT_Temp -> (junction 15270)
        (junction 15270) -> OpCl_doors.OpCl_0.Opening0.Stop_Opening [order 2]
        (junction 20169) -> (junction 15270) [order 2]
        (junction 22113) -> OpCl_doors.OpCl_0.Opening0.Timer_open [order 1] : [not(OBS)]
        OpCl_doors.OpCl_0.Opening0.Opening1 -> (junction 15274)
        OpCl_doors.OpCl_0.Opening0.People_IN -> OpCl_doors.OpCl_0.Opening0.People_OUT
        OpCl_doors.OpCl_0.Opening0.People_OUT -> (junction 22113)
        (junction 22113) -> (junction 15272) [order 2]
        (junction 15272) -> OpCl_doors.OpCl_0.Opening0.BUTT_Temp1 [order 1] : [not(FLAG==4)]
        OpCl_doors.OpCl_0.Opening0.BUTT_Temp1 -> (junction 15275)
        (junction 15275) -> OpCl_doors.OpCl_0.Opening0.Opening1 [order 1] : [not(PA0)]
        (default) -> OpCl_doors.OpCl_0.Opening0.People_IN
        (junction 15272) -> (junction 15275) [order 2]
        (junction 15276) -> (junction 15274)
        (junction 15275) -> OpCl_doors.OpCl_0.Opening0.Stop_Opening1 [order 2]
        OpCl_doors.OpCl_0.Opening0.Stop_Opening1 -> (junction 15276)
      (default) -> (junction 9095)
      (junction 9095) -> (junction 9094) [order 1] : [FLAG_OD]
      (junction 9094) -> OpCl_doors.OpCl_0.Closing0 [order 1] : [not(SWITCH) && not(STOP) && WEIGHT<=320 && not(PS0 || P0) ]
      (junction 9095) -> OpCl_doors.OpCl_0.Opening0 [order 2]
      (junction 9094) -> OpCl_doors.OpCl_0.StopClosing [order 2]
      OpCl_doors.OpCl_0.Closing0 -> (junction 14333)
      OpCl_doors.OpCl_0.StopClosing -> (junction 14333)
      (junction 14333) -> (junction 14336)
      OpCl_doors.OpCl_0.Opening0 -> (junction 14336)
    state No_floor
    state OpCl_1
      state Closing1
        state Timer_close
          state Set_tmr
            en: Q_cl=true;
          state Set
            en:PT_cl=5;
            IN_cl=true;
          state Counting
            en:ET_cl = ET_cl + 1;
            Q_cl=false;
          (junction 15536) -> OpCl_doors.OpCl_1.Closing1.Timer_close.Set_tmr [order 1] : [ET_cl==PT_cl]
          OpCl_doors.OpCl_1.Closing1.Timer_close.Set_tmr -> (junction 15537)
          (default) -> OpCl_doors.OpCl_1.Closing1.Timer_close.Set
          OpCl_doors.OpCl_1.Closing1.Timer_close.Counting -> (junction 15536)
          (junction 15536) -> (junction 15537) [order 2]
          OpCl_doors.OpCl_1.Closing1.Timer_close.Set -> (junction 15538)
          (junction 15538) -> OpCl_doors.OpCl_1.Closing1.Timer_close.Counting [order 1] : [ET_cl<PT_cl]
          (junction 15538) -> (junction 15537) [order 2]
        state BUTT_Temp
          state Butt_temp0
            en: BUT_TEMP = 0;
            FLAG_BT=true;
            LPC0=true;
          state Butt_temp1
            en: BUT_TEMP = 1;
            FLAG_BT=true;
            LPC1=true;
          state Butt_temp2
            en: BUT_TEMP = 2;
            FLAG_BT=true;
            LPC2=true;
          state Butt_temp3
            en: BUT_TEMP = 3;
            FLAG_BT=true;
            LPC3=true;
          (default) -> (junction 15551)
          (junction 15551) -> (junction 15552) [order 1] : [not(FLAG_BT)]
          (junction 15552) -> OpCl_doors.OpCl_1.Closing1.BUTT_Temp.Butt_temp0 [order 1] : [P0]
          OpCl_doors.OpCl_1.Closing1.BUTT_Temp.Butt_temp0 -> (junction 15553)
          (junction 15551) -> (junction 15560) [order 2]
          (junction 15552) -> (junction 15555) [order 2]
          (junction 15553) -> (junction 15554)
          (junction 15555) -> OpCl_doors.OpCl_1.Closing1.BUTT_Temp.Butt_temp1 [order 1] : [P1]
          OpCl_doors.OpCl_1.Closing1.BUTT_Temp.Butt_temp1 -> (junction 15554)
          (junction 15555) -> (junction 15556) [order 2]
          (junction 15554) -> (junction 15557)
          (junction 15556) -> OpCl_doors.OpCl_1.Closing1.BUTT_Temp.Butt_temp2 [order 1] : [P2]
          OpCl_doors.OpCl_1.Closing1.BUTT_Temp.Butt_temp2 -> (junction 15557)
          (junction 15556) -> (junction 15558) [order 2]
          (junction 15557) -> (junction 15559)
          (junction 15558) -> OpCl_doors.OpCl_1.Closing1.BUTT_Temp.Butt_temp3 [order 1] : [P3]
          OpCl_doors.OpCl_1.Closing1.BUTT_Temp.Butt_temp3 -> (junction 15559)
          (junction 15558) -> (junction 15561) [order 2]
          (junction 15559) -> (junction 15562)
          (junction 15560) -> (junction 15561)
          (junction 15561) -> (junction 15562)
        state Closing
          en: CP1=Q_cl;
        state Stop_Closing
          en: CP1=false;
          LPS0=false;
          LPS1=false;
          LPD1=false;
          LPS2=false;
          LPD2=false;
          LPD3=false;
          FLAG_OD=false;
          OBS=false;
          ET_cl=0;
          IN_cl=false;
        state Flag_position
          en:FLAG=2;
          FLAG_BT=false;
          BUTTON=BUT_TEMP;
        state Closing1
          en:CP1=true;
        state Flag_floor
          en: FLAG=1;
        state Stop_Closing1
          en:CP1=false;
        OpCl_doors.OpCl_1.Closing1.Closing -> OpCl_doors.OpCl_1.Closing1.BUTT_Temp
        (default) -> (junction 15503)
        (junction 15503) -> OpCl_doors.OpCl_1.Closing1.Timer_close [order 1] : [not(FLAG==0) && not(FLAG==4)]
        OpCl_doors.OpCl_1.Closing1.Timer_close -> (junction 15504)
        OpCl_doors.OpCl_1.Closing1.BUTT_Temp -> (junction 15505)
        (junction 15504) -> OpCl_doors.OpCl_1.Closing1.Closing [order 1] : [not(PC1)]
        (junction 15503) -> (junction 15507) [order 2]
        (junction 15504) -> OpCl_doors.OpCl_1.Closing1.Stop_Closing [order 2]
        (junction 15505) -> (junction 15509)
        OpCl_doors.OpCl_1.Closing1.Stop_Closing -> (junction 15506)
        (junction 15506) -> OpCl_doors.OpCl_1.Closing1.Flag_position [order 1] : [FLAG_BT]
        (junction 15506) -> OpCl_doors.OpCl_1.Closing1.Flag_floor [order 2]
        OpCl_doors.OpCl_1.Closing1.Flag_position -> (junction 15510)
        (junction 15507) -> OpCl_doors.OpCl_1.Closing1.Closing1 [order 1] : [not(PC1)]
        OpCl_doors.OpCl_1.Closing1.Closing1 -> (junction 15508)
        (junction 15507) -> OpCl_doors.OpCl_1.Closing1.Stop_Closing1 [order 2]
        (junction 15508) -> (junction 15511)
        OpCl_doors.OpCl_1.Closing1.Flag_floor -> (junction 15510)
        (junction 15510) -> (junction 15509)
        (junction 15509) -> (junction 15512)
        OpCl_doors.OpCl_1.Closing1.Stop_Closing1 -> (junction 15511)
        (junction 15511) -> (junction 15512)
      state StopClosing
        en: CP1=false;
        FLAG_OD=false;
      state Opening1
        state Opening
          en:AP1=Q_op;
        state Stop_Opening
          en:AP1=false;
          FLAG_OD=true;
          OBS=true;
          IN_op=false;
          ET_op=0;
        state Timer_open
          state Set_tmr
            en: Q_op=true;
          state Set
            en:PT_op=2;
            IN_op=true;
          state Counting
            en:ET_op = ET_op + 1;
            Q_op=false;
          (junction 20206) -> OpCl_doors.OpCl_1.Opening1.Timer_open.Set_tmr [order 1] : [ET_op==PT_op]
          OpCl_doors.OpCl_1.Opening1.Timer_open.Set_tmr -> (junction 20207)
          (default) -> OpCl_doors.OpCl_1.Opening1.Timer_open.Set
          OpCl_doors.OpCl_1.Opening1.Timer_open.Counting -> (junction 20206)
          (junction 20206) -> (junction 20207) [order 2]
          OpCl_doors.OpCl_1.Opening1.Timer_open.Set -> (junction 20208)
          (junction 20208) -> OpCl_doors.OpCl_1.Opening1.Timer_open.Counting [order 1] : [ET_op<PT_op]
          (junction 20208) -> (junction 20207) [order 2]
        state BUTT_Temp
          state Butt_temp0
            en: BUT_TEMP = 0;
            FLAG_BT=true;
            LPC0=true;
          state Butt_temp1
            en: BUT_TEMP = 1;
            FLAG_BT=true;
            LPC1=true;
          state Butt_temp2
            en: BUT_TEMP = 2;
            FLAG_BT=true;
            LPC2=true;
          state Butt_temp3
            en: BUT_TEMP = 3;
            FLAG_BT=true;
            LPC3=true;
          (default) -> (junction 20221)
          (junction 20221) -> (junction 20222) [order 1] : [not(FLAG_BT)]
          (junction 20222) -> OpCl_doors.OpCl_1.Opening1.BUTT_Temp.Butt_temp0 [order 1] : [P0]
          OpCl_doors.OpCl_1.Opening1.BUTT_Temp.Butt_temp0 -> (junction 20223)
          (junction 20222) -> (junction 20225) [order 2]
          (junction 20223) -> (junction 20224)
          (junction 20221) -> (junction 20232) [order 2]
          OpCl_doors.OpCl_1.Opening1.BUTT_Temp.Butt_temp1 -> (junction 20224)
          (junction 20225) -> OpCl_doors.OpCl_1.Opening1.BUTT_Temp.Butt_temp1 [order 1] : [P1]
          (junction 20224) -> (junction 20227)
          (junction 20225) -> (junction 20226) [order 2]
          (junction 20226) -> OpCl_doors.OpCl_1.Opening1.BUTT_Temp.Butt_temp2 [order 1] : [P2]
          OpCl_doors.OpCl_1.Opening1.BUTT_Temp.Butt_temp2 -> (junction 20227)
          (junction 20226) -> (junction 20228) [order 2]
          (junction 20227) -> (junction 20229)
          (junction 20228) -> OpCl_doors.OpCl_1.Opening1.BUTT_Temp.Butt_temp3 [order 1] : [P3]
          OpCl_doors.OpCl_1.Opening1.BUTT_Temp.Butt_temp3 -> (junction 20229)
          (junction 20229) -> (junction 20231)
          (junction 20228) -> (junction 20230) [order 2]
          (junction 20231) -> (junction 20230)
          (junction 20230) -> (junction 20233)
          (junction 20232) -> (junction 20233)
        state BUTT_Temp1
          state Butt_temp0
            en: BUT_TEMP = 0;
            FLAG_BT=true;
            LPC0=true;
          state Butt_temp1
            en: BUT_TEMP = 1;
            FLAG_BT=true;
            LPC1=true;
          state Butt_temp2
            en: BUT_TEMP = 2;
            FLAG_BT=true;
            LPC2=true;
          state Butt_temp3
            en: BUT_TEMP = 3;
            FLAG_BT=true;
            LPC3=true;
          (default) -> (junction 20261)
          (junction 20261) -> (junction 20262) [order 1] : [not(FLAG_BT)]
          (junction 20262) -> OpCl_doors.OpCl_1.Opening1.BUTT_Temp1.Butt_temp0 [order 1] : [P0]
          OpCl_doors.OpCl_1.Opening1.BUTT_Temp1.Butt_temp0 -> (junction 20263)
          (junction 20262) -> (junction 20265) [order 2]
          (junction 20263) -> (junction 20264)
          (junction 20261) -> (junction 20272) [order 2]
          OpCl_doors.OpCl_1.Opening1.BUTT_Temp1.Butt_temp1 -> (junction 20264)
          (junction 20265) -> OpCl_doors.OpCl_1.Opening1.BUTT_Temp1.Butt_temp1 [order 1] : [P1]
          (junction 20264) -> (junction 20267)
          (junction 20265) -> (junction 20266) [order 2]
          (junction 20266) -> OpCl_doors.OpCl_1.Opening1.BUTT_Temp1.Butt_temp2 [order 1] : [P2]
          OpCl_doors.OpCl_1.Opening1.BUTT_Temp1.Butt_temp2 -> (junction 20267)
          (junction 20266) -> (junction 20268) [order 2]
          (junction 20267) -> (junction 20269)
          (junction 20268) -> OpCl_doors.OpCl_1.Opening1.BUTT_Temp1.Butt_temp3 [order 1] : [P3]
          OpCl_doors.OpCl_1.Opening1.BUTT_Temp1.Butt_temp3 -> (junction 20269)
          (junction 20269) -> (junction 20271)
          (junction 20268) -> (junction 20270) [order 2]
          (junction 20271) -> (junction 20270)
          (junction 20270) -> (junction 20273)
          (junction 20272) -> (junction 20273)
        state Opening1
          en:AP1=true;
        state People_IN
          state Check_People_IN
            en:
            COUNTER_IN=false;
          state Ready_IN
            en:
            IN_DEL_IN=false;
            ET_DEL_IN=0;
          state People_KID_IN
            en:
            WEIGHT=WEIGHT+30;
            KIDS=KIDS+1;
          state DELAY_IN
            state Set_tmr
              en:
              Q_DEL_IN=true;
            state Counting
              en:
              ET_DEL_IN = ET_DEL_IN + 1;
              Q_DEL_IN=false;
            state Set
              en:
              IN_DEL_IN=true;
              PT_DEL_IN=0.05;
            (junction 20357) -> OpCl_doors.OpCl_1.Opening1.People_IN.DELAY_IN.Set_tmr [order 1] : [ET_DEL_IN==PT_DEL_IN]
            OpCl_doors.OpCl_1.Opening1.People_IN.DELAY_IN.Set_tmr -> (junction 20358)
            OpCl_doors.OpCl_1.Opening1.People_IN.DELAY_IN.Counting -> (junction 20357)
            (junction 20357) -> (junction 20358) [order 2]
            (default) -> OpCl_doors.OpCl_1.Opening1.People_IN.DELAY_IN.Set
            OpCl_doors.OpCl_1.Opening1.People_IN.DELAY_IN.Set -> (junction 20359)
            (junction 20359) -> OpCl_doors.OpCl_1.Opening1.People_IN.DELAY_IN.Counting [order 1] : [ET_DEL_IN<PT_DEL_IN]
            (junction 20359) -> (junction 20358) [order 2]
          state People_WOMAN_IN
            en:
            WEIGHT=WEIGHT+55;
            WOMEN=WOMEN+1;
          state People_MAN_IN
            en:
            WEIGHT=WEIGHT+75;
            MEN=MEN+1;
          state People_FATGUY_IN
            en:
            WEIGHT=WEIGHT+100;
            FATGUYS=FATGUYS+1;
          state Re_Ready_IN
            en:
            COUNTER_IN=true;
          OpCl_doors.OpCl_1.Opening1.People_IN.Check_People_IN -> (junction 20302)
          (junction 20302) -> OpCl_doors.OpCl_1.Opening1.People_IN.People_KID_IN [order 1] : [KID_IN]
          OpCl_doors.OpCl_1.Opening1.People_IN.People_KID_IN -> (junction 20303)
          OpCl_doors.OpCl_1.Opening1.People_IN.DELAY_IN -> (junction 20304)
          (junction 20304) -> OpCl_doors.OpCl_1.Opening1.People_IN.Ready_IN [order 1] : [Q_DEL_IN]
          (default) -> OpCl_doors.OpCl_1.Opening1.People_IN.DELAY_IN
          OpCl_doors.OpCl_1.Opening1.People_IN.Ready_IN -> (junction 20305)
          (junction 20305) -> OpCl_doors.OpCl_1.Opening1.People_IN.Check_People_IN [order 1] : [COUNTER_IN]
          (junction 20302) -> (junction 20307) [order 2]
          (junction 20303) -> (junction 20306)
          (junction 20304) -> (junction 20316) [order 2]
          (junction 20305) -> (junction 20315) [order 2]
          (junction 20307) -> OpCl_doors.OpCl_1.Opening1.People_IN.People_WOMAN_IN [order 1] : [WOMAN_IN]
          OpCl_doors.OpCl_1.Opening1.People_IN.People_WOMAN_IN -> (junction 20306)
          (junction 20307) -> (junction 20308) [order 2]
          (junction 20306) -> (junction 20309)
          (junction 20308) -> OpCl_doors.OpCl_1.Opening1.People_IN.People_MAN_IN [order 1] : [MAN_IN]
          OpCl_doors.OpCl_1.Opening1.People_IN.People_MAN_IN -> (junction 20309)
          (junction 20308) -> (junction 20310) [order 2]
          (junction 20309) -> (junction 20311)
          (junction 20310) -> OpCl_doors.OpCl_1.Opening1.People_IN.People_FATGUY_IN [order 1] : [FATGUY_IN]
          OpCl_doors.OpCl_1.Opening1.People_IN.People_FATGUY_IN -> (junction 20311)
          (junction 20310) -> (junction 20312) [order 2]
          (junction 20311) -> (junction 20313)
          (junction 20312) -> (junction 20313)
          (junction 20313) -> (junction 20314)
          (junction 20315) -> (junction 20314)
          (junction 20314) -> (junction 20317)
          (junction 20316) -> (junction 20317)
          (junction 20317) -> (junction 20318)
          (junction 20318) -> OpCl_doors.OpCl_1.Opening1.People_IN.Re_Ready_IN [order 1] : [not(KID_IN|| WOMAN_IN || MAN_IN || FATGUY_IN)]
          (junction 20318) -> (junction 20319) [order 2]
          OpCl_doors.OpCl_1.Opening1.People_IN.Re_Ready_IN -> (junction 20319)
        state People_OUT
          state Ready_OUT
            en:
            IN_DEL_OUT=false;
            ET_DEL_OUT=0;
          state Check_People_OUT
            en:
            COUNTER_OUT=false;
          state People_KID_OUT
            en:
            WEIGHT=WEIGHT-30;
            KIDS=KIDS-1;
          state DELAY_OUT
            state Set_tmr
              en:
              Q_DEL_OUT=true;
            state Counting
              en:
              ET_DEL_OUT = ET_DEL_OUT + 1;
              Q_DEL_OUT=false;
            state Set
              en:
              IN_DEL_OUT=true;
              PT_DEL_OUT=0.05;
            (junction 20431) -> OpCl_doors.OpCl_1.Opening1.People_OUT.DELAY_OUT.Set_tmr [order 1] : [ET_DEL_OUT==PT_DEL_OUT]
            OpCl_doors.OpCl_1.Opening1.People_OUT.DELAY_OUT.Set_tmr -> (junction 20432)
            OpCl_doors.OpCl_1.Opening1.People_OUT.DELAY_OUT.Counting -> (junction 20431)
            (junction 20431) -> (junction 20432) [order 2]
            (default) -> OpCl_doors.OpCl_1.Opening1.People_OUT.DELAY_OUT.Set
            OpCl_doors.OpCl_1.Opening1.People_OUT.DELAY_OUT.Set -> (junction 20433)
            (junction 20433) -> OpCl_doors.OpCl_1.Opening1.People_OUT.DELAY_OUT.Counting [order 1] : [ET_DEL_OUT<PT_DEL_OUT]
            (junction 20433) -> (junction 20432) [order 2]
          state People_WOMAN_OUT
            en:
            WEIGHT=WEIGHT-55;
            WOMEN=WOMEN-1;
          state People_MAN_OUT
            en:
            WEIGHT=WEIGHT-75;
            MEN=MEN-1;
          state People_FATGUY_OUT
            en:
            WEIGHT=WEIGHT-100;
            FATGUYS=FATGUYS-1;
          state Re_Ready_OUT
            en:
            COUNTER_OUT=true;
          (default) -> OpCl_doors.OpCl_1.Opening1.People_OUT.DELAY_OUT
          OpCl_doors.OpCl_1.Opening1.People_OUT.DELAY_OUT -> (junction 20376)
          (junction 20376) -> OpCl_doors.OpCl_1.Opening1.People_OUT.Ready_OUT [order 1] : [Q_DEL_OUT]
          OpCl_doors.OpCl_1.Opening1.People_OUT.Ready_OUT -> (junction 20377)
          (junction 20377) -> OpCl_doors.OpCl_1.Opening1.People_OUT.Check_People_OUT [order 1] : [COUNTER_OUT]
          OpCl_doors.OpCl_1.Opening1.People_OUT.Check_People_OUT -> (junction 20378)
          (junction 20378) -> OpCl_doors.OpCl_1.Opening1.People_OUT.People_KID_OUT [order 1] : [KID_OUT && KIDS>0 ]
          OpCl_doors.OpCl_1.Opening1.People_OUT.People_KID_OUT -> (junction 20379)
          (junction 20376) -> (junction 20390) [order 2]
          (junction 20377) -> (junction 20388) [order 2]
          (junction 20378) -> (junction 20380) [order 2]
          (junction 20379) -> (junction 20381)
          (junction 20380) -> OpCl_doors.OpCl_1.Opening1.People_OUT.People_WOMAN_OUT [order 1] : [WOMAN_OUT && WOMEN>0]
          OpCl_doors.OpCl_1.Opening1.People_OUT.People_WOMAN_OUT -> (junction 20381)
          (junction 20380) -> (junction 20383) [order 2]
          (junction 20381) -> (junction 20382)
          (junction 20383) -> OpCl_doors.OpCl_1.Opening1.People_OUT.People_MAN_OUT [order 1] : [MAN_OUT && MEN>0]
          OpCl_doors.OpCl_1.Opening1.People_OUT.People_MAN_OUT -> (junction 20382)
          (junction 20383) -> (junction 20384) [order 2]
          (junction 20382) -> (junction 20385)
          (junction 20384) -> OpCl_doors.OpCl_1.Opening1.People_OUT.People_FATGUY_OUT [order 1] : [FATGUY_OUT && FATGUYS>0]
          OpCl_doors.OpCl_1.Opening1.People_OUT.People_FATGUY_OUT -> (junction 20385)
          (junction 20384) -> (junction 20387) [order 2]
          (junction 20385) -> (junction 20386)
          (junction 20387) -> (junction 20386)
          (junction 20386) -> (junction 20389)
          (junction 20388) -> (junction 20389)
          (junction 20389) -> (junction 20391)
          (junction 20390) -> (junction 20391)
          (junction 20391) -> (junction 20392)
          (junction 20392) -> OpCl_doors.OpCl_1.Opening1.People_OUT.Re_Ready_OUT [order 1] : [not(KID_OUT || WOMAN_OUT || MAN_OUT || FATGUY_OUT)]
          (junction 20392) -> (junction 20393) [order 2]
          OpCl_doors.OpCl_1.Opening1.People_OUT.Re_Ready_OUT -> (junction 20393)
        state Stop_Opening1
          en: AP1=false;
          FLAG_OD=true;
          IN_cl=false;
          ET_cl=0;
        OpCl_doors.OpCl_1.Opening1.Opening -> (junction 20175)
        (junction 20175) -> (junction 20174)
        OpCl_doors.OpCl_1.Opening1.Stop_Opening -> (junction 20175)
        (junction 20174) -> (junction 20178)
        (junction 20177) -> OpCl_doors.OpCl_1.Opening1.Opening [order 1] : [not(PA1)]
        (junction 20176) -> OpCl_doors.OpCl_1.Opening1.BUTT_Temp [order 1] : [not(FLAG==4)]
        OpCl_doors.OpCl_1.Opening1.BUTT_Temp -> (junction 20177)
        (junction 20177) -> OpCl_doors.OpCl_1.Opening1.Stop_Opening [order 2]
        OpCl_doors.OpCl_1.Opening1.Timer_open -> (junction 20176)
        (junction 20176) -> (junction 20177) [order 2]
        (junction 22115) -> OpCl_doors.OpCl_1.Opening1.Timer_open [order 1] : [not(OBS)]
        OpCl_doors.OpCl_1.Opening1.Opening1 -> (junction 20178)
        (junction 20179) -> OpCl_doors.OpCl_1.Opening1.Opening1 [order 1] : [not(PA1)]
        OpCl_doors.OpCl_1.Opening1.BUTT_Temp1 -> (junction 20179)
        OpCl_doors.OpCl_1.Opening1.People_IN -> OpCl_doors.OpCl_1.Opening1.People_OUT
        OpCl_doors.OpCl_1.Opening1.People_OUT -> (junction 22115)
        (junction 22115) -> (junction 20180) [order 2]
        (junction 20180) -> OpCl_doors.OpCl_1.Opening1.BUTT_Temp1 [order 1] : [not(FLAG==4)]
        (default) -> OpCl_doors.OpCl_1.Opening1.People_IN
        (junction 20180) -> (junction 20179) [order 2]
        (junction 20181) -> (junction 20178)
        (junction 20179) -> OpCl_doors.OpCl_1.Opening1.Stop_Opening1 [order 2]
        OpCl_doors.OpCl_1.Opening1.Stop_Opening1 -> (junction 20181)
      (default) -> (junction 15489)
      (junction 15489) -> (junction 15490) [order 1] : [FLAG_OD]
      (junction 15490) -> OpCl_doors.OpCl_1.Closing1 [order 1] : [not(SWITCH) && not(STOP) && WEIGHT<=320 && not(PS1 || PD1 || P1) ]
      (junction 15489) -> OpCl_doors.OpCl_1.Opening1 [order 2]
      (junction 15490) -> OpCl_doors.OpCl_1.StopClosing [order 2]
      OpCl_doors.OpCl_1.Closing1 -> (junction 15491)
      OpCl_doors.OpCl_1.StopClosing -> (junction 15491)
      (junction 15491) -> (junction 15492)
      OpCl_doors.OpCl_1.Opening1 -> (junction 15492)
    state OpCl_2
      state Closing2
        state Timer_close
          state Set_tmr
            en: Q_cl=true;
          state Set
            en:PT_cl=5;
            IN_cl=true;
          state Counting
            en:ET_cl = ET_cl + 1;
            Q_cl=false;
          (junction 15864) -> OpCl_doors.OpCl_2.Closing2.Timer_close.Set_tmr [order 1] : [ET_cl==PT_cl]
          OpCl_doors.OpCl_2.Closing2.Timer_close.Set_tmr -> (junction 15865)
          (default) -> OpCl_doors.OpCl_2.Closing2.Timer_close.Set
          OpCl_doors.OpCl_2.Closing2.Timer_close.Counting -> (junction 15864)
          (junction 15864) -> (junction 15865) [order 2]
          OpCl_doors.OpCl_2.Closing2.Timer_close.Set -> (junction 15866)
          (junction 15866) -> OpCl_doors.OpCl_2.Closing2.Timer_close.Counting [order 1] : [ET_cl<PT_cl]
          (junction 15866) -> (junction 15865) [order 2]
        state BUTT_Temp
          state Butt_temp0
            en: BUT_TEMP = 0;
            FLAG_BT=true;
            LPC0=true;
          state Butt_temp1
            en: BUT_TEMP = 1;
            FLAG_BT=true;
            LPC1=true;
          state Butt_temp2
            en: BUT_TEMP = 2;
            FLAG_BT=true;
            LPC2=true;
          state Butt_temp3
            en: BUT_TEMP = 3;
            FLAG_BT=true;
            LPC3=true;
          (default) -> (junction 15879)
          (junction 15879) -> (junction 15880) [order 1] : [not(FLAG_BT)]
          (junction 15880) -> OpCl_doors.OpCl_2.Closing2.BUTT_Temp.Butt_temp0 [order 1] : [P0]
          OpCl_doors.OpCl_2.Closing2.BUTT_Temp.Butt_temp0 -> (junction 15881)
          (junction 15879) -> (junction 15888) [order 2]
          (junction 15880) -> (junction 15883) [order 2]
          (junction 15881) -> (junction 15882)
          (junction 15883) -> OpCl_doors.OpCl_2.Closing2.BUTT_Temp.Butt_temp1 [order 1] : [P1]
          OpCl_doors.OpCl_2.Closing2.BUTT_Temp.Butt_temp1 -> (junction 15882)
          (junction 15883) -> (junction 15884) [order 2]
          (junction 15882) -> (junction 15885)
          (junction 15884) -> OpCl_doors.OpCl_2.Closing2.BUTT_Temp.Butt_temp2 [order 1] : [P2]
          OpCl_doors.OpCl_2.Closing2.BUTT_Temp.Butt_temp2 -> (junction 15885)
          (junction 15884) -> (junction 15886) [order 2]
          (junction 15885) -> (junction 15887)
          (junction 15886) -> OpCl_doors.OpCl_2.Closing2.BUTT_Temp.Butt_temp3 [order 1] : [P3]
          OpCl_doors.OpCl_2.Closing2.BUTT_Temp.Butt_temp3 -> (junction 15887)
          (junction 15886) -> (junction 15889) [order 2]
          (junction 15887) -> (junction 15890)
          (junction 15888) -> (junction 15889)
          (junction 15889) -> (junction 15890)
        state Closing
          en: CP2=Q_cl;
        state Stop_Closing
          en: CP2=false;
          LPS0=false;
          LPS1=false;
          LPD1=false;
          LPS2=false;
          LPD2=false;
          LPD3=false;
          FLAG_OD=false;
          OBS=false;
          ET_cl=0;
          IN_cl=false;
        state Flag_position
          en:FLAG=2;
          FLAG_BT=false;
          BUTTON=BUT_TEMP;
        state Closing1
          en:CP2=true;
        state Flag_floor
          en: FLAG=1;
        state Stop_Closing1
          en:CP2=false;
        OpCl_doors.OpCl_2.Closing2.Closing -> OpCl_doors.OpCl_2.Closing2.BUTT_Temp
        (default) -> (junction 15831)
        (junction 15831) -> OpCl_doors.OpCl_2.Closing2.Timer_close [order 1] : [not(FLAG==0) && not(FLAG==4)]
        OpCl_doors.OpCl_2.Closing2.Timer_close -> (junction 15832)
        OpCl_doors.OpCl_2.Closing2.BUTT_Temp -> (junction 15833)
        (junction 15832) -> OpCl_doors.OpCl_2.Closing2.Closing [order 1] : [not(PC2)]
        (junction 15831) -> (junction 15835) [order 2]
        (junction 15832) -> OpCl_doors.OpCl_2.Closing2.Stop_Closing [order 2]
        (junction 15833) -> (junction 15837)
        OpCl_doors.OpCl_2.Closing2.Stop_Closing -> (junction 15834)
        (junction 15834) -> OpCl_doors.OpCl_2.Closing2.Flag_position [order 1] : [FLAG_BT]
        (junction 15834) -> OpCl_doors.OpCl_2.Closing2.Flag_floor [order 2]
        OpCl_doors.OpCl_2.Closing2.Flag_position -> (junction 15838)
        (junction 15835) -> OpCl_doors.OpCl_2.Closing2.Closing1 [order 1] : [not(PC2)]
        OpCl_doors.OpCl_2.Closing2.Closing1 -> (junction 15836)
        (junction 15835) -> OpCl_doors.OpCl_2.Closing2.Stop_Closing1 [order 2]
        (junction 15836) -> (junction 15839)
        OpCl_doors.OpCl_2.Closing2.Flag_floor -> (junction 15838)
        (junction 15838) -> (junction 15837)
        (junction 15837) -> (junction 15840)
        OpCl_doors.OpCl_2.Closing2.Stop_Closing1 -> (junction 15839)
        (junction 15839) -> (junction 15840)
      state StopClosing
        en: CP2=false;
        FLAG_OD=false;
      state Opening2
        state Opening
          en:AP2=Q_op;
        state Stop_Opening
          en:AP2=false;
          FLAG_OD=true;
          OBS=true;
          IN_op=false;
          ET_op=0;
        state Timer_open
          state Set_tmr
            en: Q_op=true;
          state Set
            en:PT_op=2;
            IN_op=true;
          state Counting
            en:ET_op = ET_op + 1;
            Q_op=false;
          (junction 20483) -> OpCl_doors.OpCl_2.Opening2.Timer_open.Set_tmr [order 1] : [ET_op==PT_op]
          OpCl_doors.OpCl_2.Opening2.Timer_open.Set_tmr -> (junction 20484)
          (default) -> OpCl_doors.OpCl_2.Opening2.Timer_open.Set
          OpCl_doors.OpCl_2.Opening2.Timer_open.Counting -> (junction 20483)
          (junction 20483) -> (junction 20484) [order 2]
          OpCl_doors.OpCl_2.Opening2.Timer_open.Set -> (junction 20485)
          (junction 20485) -> OpCl_doors.OpCl_2.Opening2.Timer_open.Counting [order 1] : [ET_op<PT_op]
          (junction 20485) -> (junction 20484) [order 2]
        state BUTT_Temp
          state Butt_temp0
            en: BUT_TEMP = 0;
            FLAG_BT=true;
            LPC0=true;
          state Butt_temp1
            en: BUT_TEMP = 1;
            FLAG_BT=true;
            LPC1=true;
          state Butt_temp2
            en: BUT_TEMP = 2;
            FLAG_BT=true;
            LPC2=true;
          state Butt_temp3
            en: BUT_TEMP = 3;
            FLAG_BT=true;
            LPC3=true;
          (default) -> (junction 20498)
          (junction 20498) -> (junction 20499) [order 1] : [not(FLAG_BT)]
          (junction 20499) -> OpCl_doors.OpCl_2.Opening2.BUTT_Temp.Butt_temp0 [order 1] : [P0]
          OpCl_doors.OpCl_2.Opening2.BUTT_Temp.Butt_temp0 -> (junction 20500)
          (junction 20499) -> (junction 20502) [order 2]
          (junction 20500) -> (junction 20501)
          (junction 20498) -> (junction 20509) [order 2]
          OpCl_doors.OpCl_2.Opening2.BUTT_Temp.Butt_temp1 -> (junction 20501)
          (junction 20502) -> OpCl_doors.OpCl_2.Opening2.BUTT_Temp.Butt_temp1 [order 1] : [P1]
          (junction 20501) -> (junction 20504)
          (junction 20502) -> (junction 20503) [order 2]
          (junction 20503) -> OpCl_doors.OpCl_2.Opening2.BUTT_Temp.Butt_temp2 [order 1] : [P2]
          OpCl_doors.OpCl_2.Opening2.BUTT_Temp.Butt_temp2 -> (junction 20504)
          (junction 20503) -> (junction 20505) [order 2]
          (junction 20504) -> (junction 20506)
          (junction 20505) -> OpCl_doors.OpCl_2.Opening2.BUTT_Temp.Butt_temp3 [order 1] : [P3]
          OpCl_doors.OpCl_2.Opening2.BUTT_Temp.Butt_temp3 -> (junction 20506)
          (junction 20506) -> (junction 20508)
          (junction 20505) -> (junction 20507) [order 2]
          (junction 20508) -> (junction 20507)
          (junction 20507) -> (junction 20510)
          (junction 20509) -> (junction 20510)
        state BUTT_Temp1
          state Butt_temp0
            en: BUT_TEMP = 0;
            FLAG_BT=true;
            LPC0=true;
          state Butt_temp1
            en: BUT_TEMP = 1;
            FLAG_BT=true;
            LPC1=true;
          state Butt_temp2
            en: BUT_TEMP = 2;
            FLAG_BT=true;
            LPC2=true;
          state Butt_temp3
            en: BUT_TEMP = 3;
            FLAG_BT=true;
            LPC3=true;
          (default) -> (junction 20538)
          (junction 20538) -> (junction 20539) [order 1] : [not(FLAG_BT)]
          (junction 20539) -> OpCl_doors.OpCl_2.Opening2.BUTT_Temp1.Butt_temp0 [order 1] : [P0]
          OpCl_doors.OpCl_2.Opening2.BUTT_Temp1.Butt_temp0 -> (junction 20540)
          (junction 20539) -> (junction 20542) [order 2]
          (junction 20540) -> (junction 20541)
          (junction 20538) -> (junction 20549) [order 2]
          OpCl_doors.OpCl_2.Opening2.BUTT_Temp1.Butt_temp1 -> (junction 20541)
          (junction 20542) -> OpCl_doors.OpCl_2.Opening2.BUTT_Temp1.Butt_temp1 [order 1] : [P1]
          (junction 20541) -> (junction 20544)
          (junction 20542) -> (junction 20543) [order 2]
          (junction 20543) -> OpCl_doors.OpCl_2.Opening2.BUTT_Temp1.Butt_temp2 [order 1] : [P2]
          OpCl_doors.OpCl_2.Opening2.BUTT_Temp1.Butt_temp2 -> (junction 20544)
          (junction 20543) -> (junction 20545) [order 2]
          (junction 20544) -> (junction 20546)
          (junction 20545) -> OpCl_doors.OpCl_2.Opening2.BUTT_Temp1.Butt_temp3 [order 1] : [P3]
          OpCl_doors.OpCl_2.Opening2.BUTT_Temp1.Butt_temp3 -> (junction 20546)
          (junction 20546) -> (junction 20548)
          (junction 20545) -> (junction 20547) [order 2]
          (junction 20548) -> (junction 20547)
          (junction 20547) -> (junction 20550)
          (junction 20549) -> (junction 20550)
        state Opening1
          en:AP2=true;
        state People_IN
          state Check_People_IN
            en:
            COUNTER_IN=false;
          state Ready_IN
            en:
            IN_DEL_IN=false;
            ET_DEL_IN=0;
          state People_KID_IN
            en:
            WEIGHT=WEIGHT+30;
            KIDS=KIDS+1;
          state DELAY_IN
            state Set_tmr
              en:
              Q_DEL_IN=true;
            state Counting
              en:
              ET_DEL_IN = ET_DEL_IN + 1;
              Q_DEL_IN=false;
            state Set
              en:
              IN_DEL_IN=true;
              PT_DEL_IN=0.05;
            (junction 20634) -> OpCl_doors.OpCl_2.Opening2.People_IN.DELAY_IN.Set_tmr [order 1] : [ET_DEL_IN==PT_DEL_IN]
            OpCl_doors.OpCl_2.Opening2.People_IN.DELAY_IN.Set_tmr -> (junction 20635)
            OpCl_doors.OpCl_2.Opening2.People_IN.DELAY_IN.Counting -> (junction 20634)
            (junction 20634) -> (junction 20635) [order 2]
            (default) -> OpCl_doors.OpCl_2.Opening2.People_IN.DELAY_IN.Set
            OpCl_doors.OpCl_2.Opening2.People_IN.DELAY_IN.Set -> (junction 20636)
            (junction 20636) -> OpCl_doors.OpCl_2.Opening2.People_IN.DELAY_IN.Counting [order 1] : [ET_DEL_IN<PT_DEL_IN]
            (junction 20636) -> (junction 20635) [order 2]
          state People_WOMAN_IN
            en:
            WEIGHT=WEIGHT+55;
            WOMEN=WOMEN+1;
          state People_MAN_IN
            en:
            WEIGHT=WEIGHT+75;
            MEN=MEN+1;
          state People_FATGUY_IN
            en:
            WEIGHT=WEIGHT+100;
            FATGUYS=FATGUYS+1;
          state Re_Ready_IN
            en:
            COUNTER_IN=true;
          OpCl_doors.OpCl_2.Opening2.People_IN.Check_People_IN -> (junction 20579)
          (junction 20579) -> OpCl_doors.OpCl_2.Opening2.People_IN.People_KID_IN [order 1] : [KID_IN]
          OpCl_doors.OpCl_2.Opening2.People_IN.People_KID_IN -> (junction 20580)
          OpCl_doors.OpCl_2.Opening2.People_IN.DELAY_IN -> (junction 20581)
          (junction 20581) -> OpCl_doors.OpCl_2.Opening2.People_IN.Ready_IN [order 1] : [Q_DEL_IN]
          (default) -> OpCl_doors.OpCl_2.Opening2.People_IN.DELAY_IN
          OpCl_doors.OpCl_2.Opening2.People_IN.Ready_IN -> (junction 20582)
          (junction 20582) -> OpCl_doors.OpCl_2.Opening2.People_IN.Check_People_IN [order 1] : [COUNTER_IN]
          (junction 20579) -> (junction 20584) [order 2]
          (junction 20580) -> (junction 20583)
          (junction 20581) -> (junction 20593) [order 2]
          (junction 20582) -> (junction 20592) [order 2]
          (junction 20584) -> OpCl_doors.OpCl_2.Opening2.People_IN.People_WOMAN_IN [order 1] : [WOMAN_IN]
          OpCl_doors.OpCl_2.Opening2.People_IN.People_WOMAN_IN -> (junction 20583)
          (junction 20584) -> (junction 20585) [order 2]
          (junction 20583) -> (junction 20586)
          (junction 20585) -> OpCl_doors.OpCl_2.Opening2.People_IN.People_MAN_IN [order 1] : [MAN_IN]
          OpCl_doors.OpCl_2.Opening2.People_IN.People_MAN_IN -> (junction 20586)
          (junction 20585) -> (junction 20587) [order 2]
          (junction 20586) -> (junction 20588)
          (junction 20587) -> OpCl_doors.OpCl_2.Opening2.People_IN.People_FATGUY_IN [order 1] : [FATGUY_IN]
          OpCl_doors.OpCl_2.Opening2.People_IN.People_FATGUY_IN -> (junction 20588)
          (junction 20587) -> (junction 20589) [order 2]
          (junction 20588) -> (junction 20590)
          (junction 20589) -> (junction 20590)
          (junction 20590) -> (junction 20591)
          (junction 20592) -> (junction 20591)
          (junction 20591) -> (junction 20594)
          (junction 20593) -> (junction 20594)
          (junction 20594) -> (junction 20595)
          (junction 20595) -> OpCl_doors.OpCl_2.Opening2.People_IN.Re_Ready_IN [order 1] : [not(KID_IN|| WOMAN_IN || MAN_IN || FATGUY_IN)]
          (junction 20595) -> (junction 20596) [order 2]
          OpCl_doors.OpCl_2.Opening2.People_IN.Re_Ready_IN -> (junction 20596)
        state People_OUT
          state Ready_OUT
            en:
            IN_DEL_OUT=false;
            ET_DEL_OUT=0;
          state Check_People_OUT
            en:
            COUNTER_OUT=false;
          state People_KID_OUT
            en:
            WEIGHT=WEIGHT-30;
            KIDS=KIDS-1;
          state DELAY_OUT
            state Set_tmr
              en:
              Q_DEL_OUT=true;
            state Counting
              en:
              ET_DEL_OUT = ET_DEL_OUT + 1;
              Q_DEL_OUT=false;
            state Set
              en:
              IN_DEL_OUT=true;
              PT_DEL_OUT=0.05;
            (junction 20708) -> OpCl_doors.OpCl_2.Opening2.People_OUT.DELAY_OUT.Set_tmr [order 1] : [ET_DEL_OUT==PT_DEL_OUT]
            OpCl_doors.OpCl_2.Opening2.People_OUT.DELAY_OUT.Set_tmr -> (junction 20709)
            OpCl_doors.OpCl_2.Opening2.People_OUT.DELAY_OUT.Counting -> (junction 20708)
            (junction 20708) -> (junction 20709) [order 2]
            (default) -> OpCl_doors.OpCl_2.Opening2.People_OUT.DELAY_OUT.Set
            OpCl_doors.OpCl_2.Opening2.People_OUT.DELAY_OUT.Set -> (junction 20710)
            (junction 20710) -> OpCl_doors.OpCl_2.Opening2.People_OUT.DELAY_OUT.Counting [order 1] : [ET_DEL_OUT<PT_DEL_OUT]
            (junction 20710) -> (junction 20709) [order 2]
          state People_WOMAN_OUT
            en:
            WEIGHT=WEIGHT-55;
            WOMEN=WOMEN-1;
          state People_MAN_OUT
            en:
            WEIGHT=WEIGHT-75;
            MEN=MEN-1;
          state People_FATGUY_OUT
            en:
            WEIGHT=WEIGHT-100;
            FATGUYS=FATGUYS-1;
          state Re_Ready_OUT
            en:
            COUNTER_OUT=true;
          (default) -> OpCl_doors.OpCl_2.Opening2.People_OUT.DELAY_OUT
          OpCl_doors.OpCl_2.Opening2.People_OUT.DELAY_OUT -> (junction 20653)
          (junction 20653) -> OpCl_doors.OpCl_2.Opening2.People_OUT.Ready_OUT [order 1] : [Q_DEL_OUT]
          OpCl_doors.OpCl_2.Opening2.People_OUT.Ready_OUT -> (junction 20654)
          (junction 20654) -> OpCl_doors.OpCl_2.Opening2.People_OUT.Check_People_OUT [order 1] : [COUNTER_OUT]
          OpCl_doors.OpCl_2.Opening2.People_OUT.Check_People_OUT -> (junction 20655)
          (junction 20655) -> OpCl_doors.OpCl_2.Opening2.People_OUT.People_KID_OUT [order 1] : [KID_OUT && KIDS>0 ]
          OpCl_doors.OpCl_2.Opening2.People_OUT.People_KID_OUT -> (junction 20656)
          (junction 20653) -> (junction 20667) [order 2]
          (junction 20654) -> (junction 20665) [order 2]
          (junction 20655) -> (junction 20657) [order 2]
          (junction 20656) -> (junction 20658)
          (junction 20657) -> OpCl_doors.OpCl_2.Opening2.People_OUT.People_WOMAN_OUT [order 1] : [WOMAN_OUT && WOMEN>0]
          OpCl_doors.OpCl_2.Opening2.People_OUT.People_WOMAN_OUT -> (junction 20658)
          (junction 20657) -> (junction 20660) [order 2]
          (junction 20658) -> (junction 20659)
          (junction 20660) -> OpCl_doors.OpCl_2.Opening2.People_OUT.People_MAN_OUT [order 1] : [MAN_OUT && MEN>0]
          OpCl_doors.OpCl_2.Opening2.People_OUT.People_MAN_OUT -> (junction 20659)
          (junction 20660) -> (junction 20661) [order 2]
          (junction 20659) -> (junction 20662)
          (junction 20661) -> OpCl_doors.OpCl_2.Opening2.People_OUT.People_FATGUY_OUT [order 1] : [FATGUY_OUT && FATGUYS>0]
          OpCl_doors.OpCl_2.Opening2.People_OUT.People_FATGUY_OUT -> (junction 20662)
          (junction 20661) -> (junction 20664) [order 2]
          (junction 20662) -> (junction 20663)
          (junction 20664) -> (junction 20663)
          (junction 20663) -> (junction 20666)
          (junction 20665) -> (junction 20666)
          (junction 20666) -> (junction 20668)
          (junction 20667) -> (junction 20668)
          (junction 20668) -> (junction 20669)
          (junction 20669) -> OpCl_doors.OpCl_2.Opening2.People_OUT.Re_Ready_OUT [order 1] : [not(KID_OUT || WOMAN_OUT || MAN_OUT || FATGUY_OUT)]
          (junction 20669) -> (junction 20670) [order 2]
          OpCl_doors.OpCl_2.Opening2.People_OUT.Re_Ready_OUT -> (junction 20670)
        state Stop_Opening1
          en: AP2=false;
          FLAG_OD=true;
          IN_cl=false;
          ET_cl=0;
        OpCl_doors.OpCl_2.Opening2.Opening -> (junction 20452)
        (junction 20452) -> (junction 20451)
        OpCl_doors.OpCl_2.Opening2.Stop_Opening -> (junction 20452)
        (junction 20451) -> (junction 20455)
        (junction 20454) -> OpCl_doors.OpCl_2.Opening2.Opening [order 1] : [not(PA2)]
        OpCl_doors.OpCl_2.Opening2.BUTT_Temp -> (junction 20454)
        (junction 20454) -> OpCl_doors.OpCl_2.Opening2.Stop_Opening [order 2]
        OpCl_doors.OpCl_2.Opening2.Timer_open -> (junction 20453)
        (junction 20453) -> OpCl_doors.OpCl_2.Opening2.BUTT_Temp [order 1] : [not(FLAG==4)]
        (junction 20453) -> (junction 20454) [order 2]
        (junction 20457) -> OpCl_doors.OpCl_2.Opening2.Timer_open [order 1] : [not(OBS)]
        OpCl_doors.OpCl_2.Opening2.Opening1 -> (junction 20455)
        OpCl_doors.OpCl_2.Opening2.BUTT_Temp1 -> (junction 20456)
        (junction 20456) -> OpCl_doors.OpCl_2.Opening2.Opening1 [order 1] : [not(PA2)]
        OpCl_doors.OpCl_2.Opening2.People_IN -> OpCl_doors.OpCl_2.Opening2.People_OUT
        OpCl_doors.OpCl_2.Opening2.People_OUT -> (junction 20457)
        (junction 20457) -> (junction 22118) [order 2]
        (junction 22118) -> OpCl_doors.OpCl_2.Opening2.BUTT_Temp1 [order 1] : [not(FLAG==4)]
        (default) -> OpCl_doors.OpCl_2.Opening2.People_IN
        (junction 22118) -> (junction 20456) [order 2]
        (junction 20458) -> (junction 20455)
        (junction 20456) -> OpCl_doors.OpCl_2.Opening2.Stop_Opening1 [order 2]
        OpCl_doors.OpCl_2.Opening2.Stop_Opening1 -> (junction 20458)
      (default) -> (junction 15817)
      (junction 15817) -> (junction 15818) [order 1] : [FLAG_OD]
      (junction 15818) -> OpCl_doors.OpCl_2.Closing2 [order 1] : [not(SWITCH) && not(STOP) && WEIGHT<=320 && not(PS2 || PD2 || P2) ]
      (junction 15817) -> OpCl_doors.OpCl_2.Opening2 [order 2]
      (junction 15818) -> OpCl_doors.OpCl_2.StopClosing [order 2]
      OpCl_doors.OpCl_2.Closing2 -> (junction 15819)
      OpCl_doors.OpCl_2.StopClosing -> (junction 15819)
      (junction 15819) -> (junction 15820)
      OpCl_doors.OpCl_2.Opening2 -> (junction 15820)
    state OpCl_3
      state Closing3
        state Timer_close
          state Set_tmr
            en: Q_cl=true;
          state Set
            en:PT_cl=5;
            IN_cl=true;
          state Counting
            en:ET_cl = ET_cl + 1;
            Q_cl=false;
          (junction 16192) -> OpCl_doors.OpCl_3.Closing3.Timer_close.Set_tmr [order 1] : [ET_cl==PT_cl]
          OpCl_doors.OpCl_3.Closing3.Timer_close.Set_tmr -> (junction 16193)
          (default) -> OpCl_doors.OpCl_3.Closing3.Timer_close.Set
          OpCl_doors.OpCl_3.Closing3.Timer_close.Counting -> (junction 16192)
          (junction 16192) -> (junction 16193) [order 2]
          OpCl_doors.OpCl_3.Closing3.Timer_close.Set -> (junction 16194)
          (junction 16194) -> OpCl_doors.OpCl_3.Closing3.Timer_close.Counting [order 1] : [ET_cl<PT_cl]
          (junction 16194) -> (junction 16193) [order 2]
        state BUTT_Temp
          state Butt_temp0
            en: BUT_TEMP = 0;
            FLAG_BT=true;
            LPC0=true;
          state Butt_temp1
            en: BUT_TEMP = 1;
            FLAG_BT=true;
            LPC1=true;
          state Butt_temp2
            en: BUT_TEMP = 2;
            FLAG_BT=true;
            LPC2=true;
          state Butt_temp3
            en: BUT_TEMP = 3;
            FLAG_BT=true;
            LPC3=true;
          (default) -> (junction 16207)
          (junction 16207) -> (junction 16208) [order 1] : [not(FLAG_BT)]
          (junction 16208) -> OpCl_doors.OpCl_3.Closing3.BUTT_Temp.Butt_temp0 [order 1] : [P0]
          OpCl_doors.OpCl_3.Closing3.BUTT_Temp.Butt_temp0 -> (junction 16209)
          (junction 16207) -> (junction 16216) [order 2]
          (junction 16208) -> (junction 16211) [order 2]
          (junction 16209) -> (junction 16210)
          (junction 16211) -> OpCl_doors.OpCl_3.Closing3.BUTT_Temp.Butt_temp1 [order 1] : [P1]
          OpCl_doors.OpCl_3.Closing3.BUTT_Temp.Butt_temp1 -> (junction 16210)
          (junction 16211) -> (junction 16212) [order 2]
          (junction 16210) -> (junction 16213)
          (junction 16212) -> OpCl_doors.OpCl_3.Closing3.BUTT_Temp.Butt_temp2 [order 1] : [P2]
          OpCl_doors.OpCl_3.Closing3.BUTT_Temp.Butt_temp2 -> (junction 16213)
          (junction 16212) -> (junction 16214) [order 2]
          (junction 16213) -> (junction 16215)
          (junction 16214) -> OpCl_doors.OpCl_3.Closing3.BUTT_Temp.Butt_temp3 [order 1] : [P3]
          OpCl_doors.OpCl_3.Closing3.BUTT_Temp.Butt_temp3 -> (junction 16215)
          (junction 16214) -> (junction 16217) [order 2]
          (junction 16215) -> (junction 16218)
          (junction 16216) -> (junction 16217)
          (junction 16217) -> (junction 16218)
        state Closing
          en: CP3=Q_cl;
        state Stop_Closing
          en: CP3=false;
          LPS0=false;
          LPS1=false;
          LPD1=false;
          LPS2=false;
          LPD2=false;
          LPD3=false;
          FLAG_OD=false;
          OBS=false;
          ET_cl=0;
          IN_cl=false;
        state Flag_position
          en:FLAG=2;
          FLAG_BT=false;
          BUTTON=BUT_TEMP;
        state Closing1
          en:CP3=true;
        state Flag_floor
          en: FLAG=1;
        state Stop_Closing1
          en:CP3=false;
        OpCl_doors.OpCl_3.Closing3.Closing -> OpCl_doors.OpCl_3.Closing3.BUTT_Temp
        (default) -> (junction 16159)
        (junction 16159) -> OpCl_doors.OpCl_3.Closing3.Timer_close [order 1] : [not(FLAG==0) && not(FLAG==4)]
        OpCl_doors.OpCl_3.Closing3.Timer_close -> (junction 16160)
        OpCl_doors.OpCl_3.Closing3.BUTT_Temp -> (junction 16161)
        (junction 16160) -> OpCl_doors.OpCl_3.Closing3.Closing [order 1] : [not(PC3)]
        (junction 16159) -> (junction 16163) [order 2]
        (junction 16160) -> OpCl_doors.OpCl_3.Closing3.Stop_Closing [order 2]
        (junction 16161) -> (junction 16165)
        OpCl_doors.OpCl_3.Closing3.Stop_Closing -> (junction 16162)
        (junction 16162) -> OpCl_doors.OpCl_3.Closing3.Flag_position [order 1] : [FLAG_BT]
        (junction 16162) -> OpCl_doors.OpCl_3.Closing3.Flag_floor [order 2]
        OpCl_doors.OpCl_3.Closing3.Flag_position -> (junction 16166)
        (junction 16163) -> OpCl_doors.OpCl_3.Closing3.Closing1 [order 1] : [not(PC3)]
        OpCl_doors.OpCl_3.Closing3.Closing1 -> (junction 16164)
        (junction 16163) -> OpCl_doors.OpCl_3.Closing3.Stop_Closing1 [order 2]
        (junction 16164) -> (junction 16167)
        OpCl_doors.OpCl_3.Closing3.Flag_floor -> (junction 16166)
        (junction 16166) -> (junction 16165)
        (junction 16165) -> (junction 16168)
        OpCl_doors.OpCl_3.Closing3.Stop_Closing1 -> (junction 16167)
        (junction 16167) -> (junction 16168)
      state StopClosing
        en: CP3=false;
        FLAG_OD=false;
      state Opening3
        state Opening
          en:AP3=Q_op;
        state Stop_Opening
          en:AP3=false;
          FLAG_OD=true;
          OBS=true;
          IN_op=false;
          ET_op=0;
        state Timer_open
          state Set_tmr
            en: Q_op=true;
          state Set
            en:PT_op=2;
            IN_op=true;
          state Counting
            en:ET_op = ET_op + 1;
            Q_op=false;
          (junction 20760) -> OpCl_doors.OpCl_3.Opening3.Timer_open.Set_tmr [order 1] : [ET_op==PT_op]
          OpCl_doors.OpCl_3.Opening3.Timer_open.Set_tmr -> (junction 20761)
          (default) -> OpCl_doors.OpCl_3.Opening3.Timer_open.Set
          OpCl_doors.OpCl_3.Opening3.Timer_open.Counting -> (junction 20760)
          (junction 20760) -> (junction 20761) [order 2]
          OpCl_doors.OpCl_3.Opening3.Timer_open.Set -> (junction 20762)
          (junction 20762) -> OpCl_doors.OpCl_3.Opening3.Timer_open.Counting [order 1] : [ET_op<PT_op]
          (junction 20762) -> (junction 20761) [order 2]
        state BUTT_Temp
          state Butt_temp0
            en: BUT_TEMP = 0;
            FLAG_BT=true;
            LPC0=true;
          state Butt_temp1
            en: BUT_TEMP = 1;
            FLAG_BT=true;
            LPC1=true;
          state Butt_temp2
            en: BUT_TEMP = 2;
            FLAG_BT=true;
            LPC2=true;
          state Butt_temp3
            en: BUT_TEMP = 3;
            FLAG_BT=true;
            LPC3=true;
          (default) -> (junction 20775)
          (junction 20775) -> (junction 20776) [order 1] : [not(FLAG_BT)]
          (junction 20776) -> OpCl_doors.OpCl_3.Opening3.BUTT_Temp.Butt_temp0 [order 1] : [P0]
          OpCl_doors.OpCl_3.Opening3.BUTT_Temp.Butt_temp0 -> (junction 20777)
          (junction 20776) -> (junction 20779) [order 2]
          (junction 20777) -> (junction 20778)
          (junction 20775) -> (junction 20786) [order 2]
          OpCl_doors.OpCl_3.Opening3.BUTT_Temp.Butt_temp1 -> (junction 20778)
          (junction 20779) -> OpCl_doors.OpCl_3.Opening3.BUTT_Temp.Butt_temp1 [order 1] : [P1]
          (junction 20778) -> (junction 20781)
          (junction 20779) -> (junction 20780) [order 2]
          (junction 20780) -> OpCl_doors.OpCl_3.Opening3.BUTT_Temp.Butt_temp2 [order 1] : [P2]
          OpCl_doors.OpCl_3.Opening3.BUTT_Temp.Butt_temp2 -> (junction 20781)
          (junction 20780) -> (junction 20782) [order 2]
          (junction 20781) -> (junction 20783)
          (junction 20782) -> OpCl_doors.OpCl_3.Opening3.BUTT_Temp.Butt_temp3 [order 1] : [P3]
          OpCl_doors.OpCl_3.Opening3.BUTT_Temp.Butt_temp3 -> (junction 20783)
          (junction 20783) -> (junction 20785)
          (junction 20782) -> (junction 20784) [order 2]
          (junction 20785) -> (junction 20784)
          (junction 20784) -> (junction 20787)
          (junction 20786) -> (junction 20787)
        state BUTT_Temp1
          state Butt_temp0
            en: BUT_TEMP = 0;
            FLAG_BT=true;
            LPC0=true;
          state Butt_temp1
            en: BUT_TEMP = 1;
            FLAG_BT=true;
            LPC1=true;
          state Butt_temp2
            en: BUT_TEMP = 2;
            FLAG_BT=true;
            LPC2=true;
          state Butt_temp3
            en: BUT_TEMP = 3;
            FLAG_BT=true;
            LPC3=true;
          (default) -> (junction 20815)
          (junction 20815) -> (junction 20816) [order 1] : [not(FLAG_BT)]
          (junction 20816) -> OpCl_doors.OpCl_3.Opening3.BUTT_Temp1.Butt_temp0 [order 1] : [P0]
          OpCl_doors.OpCl_3.Opening3.BUTT_Temp1.Butt_temp0 -> (junction 20817)
          (junction 20816) -> (junction 20819) [order 2]
          (junction 20817) -> (junction 20818)
          (junction 20815) -> (junction 20826) [order 2]
          OpCl_doors.OpCl_3.Opening3.BUTT_Temp1.Butt_temp1 -> (junction 20818)
          (junction 20819) -> OpCl_doors.OpCl_3.Opening3.BUTT_Temp1.Butt_temp1 [order 1] : [P1]
          (junction 20818) -> (junction 20821)
          (junction 20819) -> (junction 20820) [order 2]
          (junction 20820) -> OpCl_doors.OpCl_3.Opening3.BUTT_Temp1.Butt_temp2 [order 1] : [P2]
          OpCl_doors.OpCl_3.Opening3.BUTT_Temp1.Butt_temp2 -> (junction 20821)
          (junction 20820) -> (junction 20822) [order 2]
          (junction 20821) -> (junction 20823)
          (junction 20822) -> OpCl_doors.OpCl_3.Opening3.BUTT_Temp1.Butt_temp3 [order 1] : [P3]
          OpCl_doors.OpCl_3.Opening3.BUTT_Temp1.Butt_temp3 -> (junction 20823)
          (junction 20823) -> (junction 20825)
          (junction 20822) -> (junction 20824) [order 2]
          (junction 20825) -> (junction 20824)
          (junction 20824) -> (junction 20827)
          (junction 20826) -> (junction 20827)
        state Opening1
          en:AP3=true;
        state People_IN
          state Check_People_IN
            en:
            COUNTER_IN=false;
          state Ready_IN
            en:
            IN_DEL_IN=false;
            ET_DEL_IN=0;
          state People_KID_IN
            en:
            WEIGHT=WEIGHT+30;
            KIDS=KIDS+1;
          state DELAY_IN
            state Set_tmr
              en:
              Q_DEL_IN=true;
            state Counting
              en:
              ET_DEL_IN = ET_DEL_IN + 1;
              Q_DEL_IN=false;
            state Set
              en:
              IN_DEL_IN=true;
              PT_DEL_IN=0.05;
            (junction 20911) -> OpCl_doors.OpCl_3.Opening3.People_IN.DELAY_IN.Set_tmr [order 1] : [ET_DEL_IN==PT_DEL_IN]
            OpCl_doors.OpCl_3.Opening3.People_IN.DELAY_IN.Set_tmr -> (junction 20912)
            OpCl_doors.OpCl_3.Opening3.People_IN.DELAY_IN.Counting -> (junction 20911)
            (junction 20911) -> (junction 20912) [order 2]
            (default) -> OpCl_doors.OpCl_3.Opening3.People_IN.DELAY_IN.Set
            OpCl_doors.OpCl_3.Opening3.People_IN.DELAY_IN.Set -> (junction 20913)
            (junction 20913) -> OpCl_doors.OpCl_3.Opening3.People_IN.DELAY_IN.Counting [order 1] : [ET_DEL_IN<PT_DEL_IN]
            (junction 20913) -> (junction 20912) [order 2]
          state People_WOMAN_IN
            en:
            WEIGHT=WEIGHT+55;
            WOMEN=WOMEN+1;
          state People_MAN_IN
            en:
            WEIGHT=WEIGHT+75;
            MEN=MEN+1;
          state People_FATGUY_IN
            en:
            WEIGHT=WEIGHT+100;
            FATGUYS=FATGUYS+1;
          state Re_Ready_IN
            en:
            COUNTER_IN=true;
          OpCl_doors.OpCl_3.Opening3.People_IN.Check_People_IN -> (junction 20856)
          (junction 20856) -> OpCl_doors.OpCl_3.Opening3.People_IN.People_KID_IN [order 1] : [KID_IN]
          OpCl_doors.OpCl_3.Opening3.People_IN.People_KID_IN -> (junction 20857)
          OpCl_doors.OpCl_3.Opening3.People_IN.DELAY_IN -> (junction 20858)
          (junction 20858) -> OpCl_doors.OpCl_3.Opening3.People_IN.Ready_IN [order 1] : [Q_DEL_IN]
          (default) -> OpCl_doors.OpCl_3.Opening3.People_IN.DELAY_IN
          OpCl_doors.OpCl_3.Opening3.People_IN.Ready_IN -> (junction 20859)
          (junction 20859) -> OpCl_doors.OpCl_3.Opening3.People_IN.Check_People_IN [order 1] : [COUNTER_IN]
          (junction 20856) -> (junction 20861) [order 2]
          (junction 20857) -> (junction 20860)
          (junction 20858) -> (junction 20870) [order 2]
          (junction 20859) -> (junction 20869) [order 2]
          (junction 20861) -> OpCl_doors.OpCl_3.Opening3.People_IN.People_WOMAN_IN [order 1] : [WOMAN_IN]
          OpCl_doors.OpCl_3.Opening3.People_IN.People_WOMAN_IN -> (junction 20860)
          (junction 20861) -> (junction 20862) [order 2]
          (junction 20860) -> (junction 20863)
          (junction 20862) -> OpCl_doors.OpCl_3.Opening3.People_IN.People_MAN_IN [order 1] : [MAN_IN]
          OpCl_doors.OpCl_3.Opening3.People_IN.People_MAN_IN -> (junction 20863)
          (junction 20862) -> (junction 20864) [order 2]
          (junction 20863) -> (junction 20865)
          (junction 20864) -> OpCl_doors.OpCl_3.Opening3.People_IN.People_FATGUY_IN [order 1] : [FATGUY_IN]
          OpCl_doors.OpCl_3.Opening3.People_IN.People_FATGUY_IN -> (junction 20865)
          (junction 20864) -> (junction 20866) [order 2]
          (junction 20865) -> (junction 20867)
          (junction 20866) -> (junction 20867)
          (junction 20867) -> (junction 20868)
          (junction 20869) -> (junction 20868)
          (junction 20868) -> (junction 20871)
          (junction 20870) -> (junction 20871)
          (junction 20871) -> (junction 20872)
          (junction 20872) -> OpCl_doors.OpCl_3.Opening3.People_IN.Re_Ready_IN [order 1] : [not(KID_IN|| WOMAN_IN || MAN_IN || FATGUY_IN)]
          (junction 20872) -> (junction 20873) [order 2]
          OpCl_doors.OpCl_3.Opening3.People_IN.Re_Ready_IN -> (junction 20873)
        state People_OUT
          state Ready_OUT
            en:
            IN_DEL_OUT=false;
            ET_DEL_OUT=0;
          state Check_People_OUT
            en:
            COUNTER_OUT=false;
          state People_KID_OUT
            en:
            WEIGHT=WEIGHT-30;
            KIDS=KIDS-1;
          state DELAY_OUT
            state Set_tmr
              en:
              Q_DEL_OUT=true;
            state Counting
              en:
              ET_DEL_OUT = ET_DEL_OUT + 1;
              Q_DEL_OUT=false;
            state Set
              en:
              IN_DEL_OUT=true;
              PT_DEL_OUT=0.05;
            (junction 20985) -> OpCl_doors.OpCl_3.Opening3.People_OUT.DELAY_OUT.Set_tmr [order 1] : [ET_DEL_OUT==PT_DEL_OUT]
            OpCl_doors.OpCl_3.Opening3.People_OUT.DELAY_OUT.Set_tmr -> (junction 20986)
            OpCl_doors.OpCl_3.Opening3.People_OUT.DELAY_OUT.Counting -> (junction 20985)
            (junction 20985) -> (junction 20986) [order 2]
            (default) -> OpCl_doors.OpCl_3.Opening3.People_OUT.DELAY_OUT.Set
            OpCl_doors.OpCl_3.Opening3.People_OUT.DELAY_OUT.Set -> (junction 20987)
            (junction 20987) -> OpCl_doors.OpCl_3.Opening3.People_OUT.DELAY_OUT.Counting [order 1] : [ET_DEL_OUT<PT_DEL_OUT]
            (junction 20987) -> (junction 20986) [order 2]
          state People_WOMAN_OUT
            en:
            WEIGHT=WEIGHT-55;
            WOMEN=WOMEN-1;
          state People_MAN_OUT
            en:
            WEIGHT=WEIGHT-75;
            MEN=MEN-1;
          state People_FATGUY_OUT
            en:
            WEIGHT=WEIGHT-100;
            FATGUYS=FATGUYS-1;
          state Re_Ready_OUT
            en:
            COUNTER_OUT=true;
          (default) -> OpCl_doors.OpCl_3.Opening3.People_OUT.DELAY_OUT
          OpCl_doors.OpCl_3.Opening3.People_OUT.DELAY_OUT -> (junction 20930)
          (junction 20930) -> OpCl_doors.OpCl_3.Opening3.People_OUT.Ready_OUT [order 1] : [Q_DEL_OUT]
          OpCl_doors.OpCl_3.Opening3.People_OUT.Ready_OUT -> (junction 20931)
          (junction 20931) -> OpCl_doors.OpCl_3.Opening3.People_OUT.Check_People_OUT [order 1] : [COUNTER_OUT]
          OpCl_doors.OpCl_3.Opening3.People_OUT.Check_People_OUT -> (junction 20932)
          (junction 20932) -> OpCl_doors.OpCl_3.Opening3.People_OUT.People_KID_OUT [order 1] : [KID_OUT && KIDS>0 ]
          OpCl_doors.OpCl_3.Opening3.People_OUT.People_KID_OUT -> (junction 20933)
          (junction 20930) -> (junction 20944) [order 2]
          (junction 20931) -> (junction 20942) [order 2]
          (junction 20932) -> (junction 20934) [order 2]
          (junction 20933) -> (junction 20935)
          (junction 20934) -> OpCl_doors.OpCl_3.Opening3.People_OUT.People_WOMAN_OUT [order 1] : [WOMAN_OUT && WOMEN>0]
          OpCl_doors.OpCl_3.Opening3.People_OUT.People_WOMAN_OUT -> (junction 20935)
          (junction 20934) -> (junction 20937) [order 2]
          (junction 20935) -> (junction 20936)
          (junction 20937) -> OpCl_doors.OpCl_3.Opening3.People_OUT.People_MAN_OUT [order 1] : [MAN_OUT && MEN>0]
          OpCl_doors.OpCl_3.Opening3.People_OUT.People_MAN_OUT -> (junction 20936)
          (junction 20937) -> (junction 20938) [order 2]
          (junction 20936) -> (junction 20939)
          (junction 20938) -> OpCl_doors.OpCl_3.Opening3.People_OUT.People_FATGUY_OUT [order 1] : [FATGUY_OUT && FATGUYS>0]
          OpCl_doors.OpCl_3.Opening3.People_OUT.People_FATGUY_OUT -> (junction 20939)
          (junction 20938) -> (junction 20941) [order 2]
          (junction 20939) -> (junction 20940)
          (junction 20941) -> (junction 20940)
          (junction 20940) -> (junction 20943)
          (junction 20942) -> (junction 20943)
          (junction 20943) -> (junction 20945)
          (junction 20944) -> (junction 20945)
          (junction 20945) -> (junction 20946)
          (junction 20946) -> OpCl_doors.OpCl_3.Opening3.People_OUT.Re_Ready_OUT [order 1] : [not(KID_OUT || WOMAN_OUT || MAN_OUT || FATGUY_OUT)]
          (junction 20946) -> (junction 20947) [order 2]
          OpCl_doors.OpCl_3.Opening3.People_OUT.Re_Ready_OUT -> (junction 20947)
        state Stop_Opening1
          en: AP3=false;
          FLAG_OD=true;
          IN_cl=false;
          ET_cl=0;
        OpCl_doors.OpCl_3.Opening3.Opening -> (junction 20729)
        (junction 20729) -> (junction 20728)
        OpCl_doors.OpCl_3.Opening3.Stop_Opening -> (junction 20729)
        (junction 20728) -> (junction 20732)
        (junction 20731) -> OpCl_doors.OpCl_3.Opening3.Opening [order 1] : [not(PA3)]
        OpCl_doors.OpCl_3.Opening3.BUTT_Temp -> (junction 20731)
        (junction 20731) -> OpCl_doors.OpCl_3.Opening3.Stop_Opening [order 2]
        OpCl_doors.OpCl_3.Opening3.Timer_open -> (junction 20730)
        (junction 20730) -> OpCl_doors.OpCl_3.Opening3.BUTT_Temp [order 1] : [not(FLAG==4)]
        (junction 20730) -> (junction 20731) [order 2]
        (junction 20734) -> OpCl_doors.OpCl_3.Opening3.Timer_open [order 1] : [not(OBS)]
        OpCl_doors.OpCl_3.Opening3.Opening1 -> (junction 20732)
        OpCl_doors.OpCl_3.Opening3.BUTT_Temp1 -> (junction 20733)
        (junction 20733) -> OpCl_doors.OpCl_3.Opening3.Opening1 [order 1] : [not(PA3)]
        OpCl_doors.OpCl_3.Opening3.People_IN -> OpCl_doors.OpCl_3.Opening3.People_OUT
        OpCl_doors.OpCl_3.Opening3.People_OUT -> (junction 20734)
        (junction 20734) -> (junction 22121) [order 2]
        (junction 22121) -> OpCl_doors.OpCl_3.Opening3.BUTT_Temp1 [order 1] : [not(FLAG==4)]
        (default) -> OpCl_doors.OpCl_3.Opening3.People_IN
        (junction 22121) -> (junction 20733) [order 2]
        (junction 20735) -> (junction 20732)
        (junction 20733) -> OpCl_doors.OpCl_3.Opening3.Stop_Opening1 [order 2]
        OpCl_doors.OpCl_3.Opening3.Stop_Opening1 -> (junction 20735)
      (default) -> (junction 16145)
      (junction 16145) -> (junction 16146) [order 1] : [FLAG_OD]
      (junction 16146) -> OpCl_doors.OpCl_3.Closing3 [order 1] : [not(SWITCH) && not(STOP) && WEIGHT<=320 && not(PD3 || P3) ]
      (junction 16145) -> OpCl_doors.OpCl_3.Opening3 [order 2]
      (junction 16146) -> OpCl_doors.OpCl_3.StopClosing [order 2]
      OpCl_doors.OpCl_3.Closing3 -> (junction 16147)
      OpCl_doors.OpCl_3.StopClosing -> (junction 16147)
      (junction 16147) -> (junction 16148)
      OpCl_doors.OpCl_3.Opening3 -> (junction 16148)
    OpCl_doors.No_floor -> (junction 9087)
    (junction 9087) -> OpCl_doors.OpCl_0 [order 1] : [FLOOR==0]
    OpCl_doors.OpCl_0 -> (junction 14346)
    (default) -> OpCl_doors.No_floor
    (junction 9087) -> (junction 14339) [order 2]
    (junction 14346) -> (junction 14348)
    (junction 14339) -> OpCl_doors.OpCl_1 [order 1] : [FLOOR==1]
    OpCl_doors.OpCl_1 -> (junction 14348)
    (junction 14339) -> (junction 14345) [order 2]
    (junction 14348) -> (junction 14349)
    (junction 14345) -> OpCl_doors.OpCl_2 [order 1] : [FLOOR==2]
    OpCl_doors.OpCl_2 -> (junction 14349)
    (junction 14345) -> (junction 14343) [order 2]
    (junction 14349) -> (junction 14350)
    (junction 14343) -> OpCl_doors.OpCl_3 [order 1] : [FLOOR==3]
    OpCl_doors.OpCl_3 -> (junction 14350)
    (junction 14343) -> (junction 14352) [order 2]
    (junction 14350) -> (junction 14351)
    (junction 14352) -> (junction 14351)
  state Emergency
    state FIRST
      en:
      LPC0=false;
      LPC1=false;
      LPC2=false;
      LPC3=false;
      FIRST=false;
    state BLK_Eme
      %BLK(LPS0)
      %BLK(LPD1)
      %BLK(LPS1)
      %BLK(LPD2)
      %BLK(LPS2)
      %BLK(LPD3)
    state Replacing
      en:
      SCENDI=true;
    state REC
      %BLK(LL)
    state OpCl
      state FLOOR_0
        en: CP0=false;
      state OpCl_0
        state Closing0
          state Timer_close
            state Set_tmr
              en: Q_cl=true;
            state Set
              en:PT_cl=5;
              IN_cl=true;
            state Counting
              en:ET_cl = ET_cl + 1;
              Q_cl=false;
            (junction 24107) -> Emergency.OpCl.OpCl_0.Closing0.Timer_close.Set_tmr [order 1] : [ET_cl==PT_cl]
            Emergency.OpCl.OpCl_0.Closing0.Timer_close.Set_tmr -> (junction 24108)
            (default) -> Emergency.OpCl.OpCl_0.Closing0.Timer_close.Set
            Emergency.OpCl.OpCl_0.Closing0.Timer_close.Counting -> (junction 24107)
            (junction 24107) -> (junction 24108) [order 2]
            Emergency.OpCl.OpCl_0.Closing0.Timer_close.Set -> (junction 24109)
            (junction 24109) -> Emergency.OpCl.OpCl_0.Closing0.Timer_close.Counting [order 1] : [ET_cl<PT_cl]
            (junction 24109) -> (junction 24108) [order 2]
          state BUTT_Temp
            state Butt_temp0
              en: BUT_TEMP = 0;
              FLAG_BT=true;
              LPC0=true;
            state Butt_temp1
              en: BUT_TEMP = 1;
              FLAG_BT=true;
              LPC1=true;
            state Butt_temp2
              en: BUT_TEMP = 2;
              FLAG_BT=true;
              LPC2=true;
            state Butt_temp3
              en: BUT_TEMP = 3;
              FLAG_BT=true;
              LPC3=true;
            (default) -> (junction 24122)
            (junction 24122) -> (junction 24123) [order 1] : [not(FLAG_BT)]
            (junction 24123) -> Emergency.OpCl.OpCl_0.Closing0.BUTT_Temp.Butt_temp0 [order 1] : [P0]
            Emergency.OpCl.OpCl_0.Closing0.BUTT_Temp.Butt_temp0 -> (junction 24124)
            (junction 24122) -> (junction 24131) [order 2]
            (junction 24123) -> (junction 24126) [order 2]
            (junction 24124) -> (junction 24125)
            (junction 24126) -> Emergency.OpCl.OpCl_0.Closing0.BUTT_Temp.Butt_temp1 [order 1] : [P1]
            Emergency.OpCl.OpCl_0.Closing0.BUTT_Temp.Butt_temp1 -> (junction 24125)
            (junction 24126) -> (junction 24127) [order 2]
            (junction 24125) -> (junction 24128)
            (junction 24127) -> Emergency.OpCl.OpCl_0.Closing0.BUTT_Temp.Butt_temp2 [order 1] : [P2]
            Emergency.OpCl.OpCl_0.Closing0.BUTT_Temp.Butt_temp2 -> (junction 24128)
            (junction 24127) -> (junction 24129) [order 2]
            (junction 24128) -> (junction 24130)
            (junction 24129) -> Emergency.OpCl.OpCl_0.Closing0.BUTT_Temp.Butt_temp3 [order 1] : [P3]
            Emergency.OpCl.OpCl_0.Closing0.BUTT_Temp.Butt_temp3 -> (junction 24130)
            (junction 24129) -> (junction 24132) [order 2]
            (junction 24130) -> (junction 24133)
            (junction 24131) -> (junction 24132)
            (junction 24132) -> (junction 24133)
          state Closing
            en: CP0=Q_cl;
          state Stop_Closing
            en: CP0=false;
            LPS0=false;
            LPS1=false;
            LPD1=false;
            LPS2=false;
            LPD2=false;
            LPD3=false;
            FLAG_OD=false;
            OBS=false;
            ET_cl=0;
            IN_cl=false;
          state Flag_position
            en:FLAG=2;
            FLAG_BT=false;
            BUTTON=BUT_TEMP;
          state Closing1
            en:CP0=true;
          state Flag_floor
            en: FLAG=1;
          state Stop_Closing1
            en:CP0=false;
          Emergency.OpCl.OpCl_0.Closing0.Closing -> Emergency.OpCl.OpCl_0.Closing0.BUTT_Temp
          (default) -> (junction 24074)
          (junction 24074) -> Emergency.OpCl.OpCl_0.Closing0.Timer_close [order 1] : [not(FLAG==0) && not(FLAG==4)]
          Emergency.OpCl.OpCl_0.Closing0.Timer_close -> (junction 24075)
          (junction 24075) -> Emergency.OpCl.OpCl_0.Closing0.Closing [order 1] : [not(PC0)]
          Emergency.OpCl.OpCl_0.Closing0.BUTT_Temp -> (junction 24076)
          (junction 24074) -> (junction 24078) [order 2]
          (junction 24075) -> Emergency.OpCl.OpCl_0.Closing0.Stop_Closing [order 2]
          (junction 24076) -> (junction 24080)
          Emergency.OpCl.OpCl_0.Closing0.Stop_Closing -> (junction 24077)
          (junction 24077) -> Emergency.OpCl.OpCl_0.Closing0.Flag_position [order 1] : [FLAG_BT]
          (junction 24077) -> Emergency.OpCl.OpCl_0.Closing0.Flag_floor [order 2]
          Emergency.OpCl.OpCl_0.Closing0.Flag_position -> (junction 24081)
          (junction 24078) -> Emergency.OpCl.OpCl_0.Closing0.Closing1 [order 1] : [not(PC0)]
          Emergency.OpCl.OpCl_0.Closing0.Closing1 -> (junction 24079)
          (junction 24078) -> Emergency.OpCl.OpCl_0.Closing0.Stop_Closing1 [order 2]
          (junction 24079) -> (junction 24082)
          Emergency.OpCl.OpCl_0.Closing0.Flag_floor -> (junction 24081)
          (junction 24081) -> (junction 24080)
          (junction 24080) -> (junction 24083)
          Emergency.OpCl.OpCl_0.Closing0.Stop_Closing1 -> (junction 24082)
          (junction 24082) -> (junction 24083)
        state StopClosing
          en: CP0=false;
          FLAG_OD=false;
        state Opening0
          state Opening
            en:AP0=Q_op;
          state Stop_Opening
            en:AP0=false;
            FLAG_OD=true;
            OBS=true;
            IN_op=false;
            ET_op=0;
          state Timer_open
            state Set_tmr
              en: Q_op=true;
            state Set
              en:PT_op=2;
              IN_op=true;
            state Counting
              en:ET_op = ET_op + 1;
              Q_op=false;
            (junction 24202) -> Emergency.OpCl.OpCl_0.Opening0.Timer_open.Set_tmr [order 1] : [ET_op==PT_op]
            Emergency.OpCl.OpCl_0.Opening0.Timer_open.Set_tmr -> (junction 24203)
            (default) -> Emergency.OpCl.OpCl_0.Opening0.Timer_open.Set
            Emergency.OpCl.OpCl_0.Opening0.Timer_open.Counting -> (junction 24202)
            (junction 24202) -> (junction 24203) [order 2]
            Emergency.OpCl.OpCl_0.Opening0.Timer_open.Set -> (junction 24204)
            (junction 24204) -> Emergency.OpCl.OpCl_0.Opening0.Timer_open.Counting [order 1] : [ET_op<PT_op]
            (junction 24204) -> (junction 24203) [order 2]
          state BUTT_Temp
            state Butt_temp0
              en: BUT_TEMP = 0;
              FLAG_BT=true;
              LPC0=true;
            state Butt_temp1
              en: BUT_TEMP = 1;
              FLAG_BT=true;
              LPC1=true;
            state Butt_temp2
              en: BUT_TEMP = 2;
              FLAG_BT=true;
              LPC2=true;
            state Butt_temp3
              en: BUT_TEMP = 3;
              FLAG_BT=true;
              LPC3=true;
            (default) -> (junction 24217)
            (junction 24217) -> (junction 24218) [order 1] : [not(FLAG_BT)]
            (junction 24218) -> Emergency.OpCl.OpCl_0.Opening0.BUTT_Temp.Butt_temp0 [order 1] : [P0]
            Emergency.OpCl.OpCl_0.Opening0.BUTT_Temp.Butt_temp0 -> (junction 24219)
            (junction 24218) -> (junction 24221) [order 2]
            (junction 24219) -> (junction 24220)
            (junction 24217) -> (junction 24228) [order 2]
            Emergency.OpCl.OpCl_0.Opening0.BUTT_Temp.Butt_temp1 -> (junction 24220)
            (junction 24221) -> Emergency.OpCl.OpCl_0.Opening0.BUTT_Temp.Butt_temp1 [order 1] : [P1]
            (junction 24220) -> (junction 24223)
            (junction 24221) -> (junction 24222) [order 2]
            (junction 24222) -> Emergency.OpCl.OpCl_0.Opening0.BUTT_Temp.Butt_temp2 [order 1] : [P2]
            Emergency.OpCl.OpCl_0.Opening0.BUTT_Temp.Butt_temp2 -> (junction 24223)
            (junction 24222) -> (junction 24224) [order 2]
            (junction 24223) -> (junction 24225)
            (junction 24224) -> Emergency.OpCl.OpCl_0.Opening0.BUTT_Temp.Butt_temp3 [order 1] : [P3]
            Emergency.OpCl.OpCl_0.Opening0.BUTT_Temp.Butt_temp3 -> (junction 24225)
            (junction 24225) -> (junction 24227)
            (junction 24224) -> (junction 24226) [order 2]
            (junction 24227) -> (junction 24226)
            (junction 24226) -> (junction 24229)
            (junction 24228) -> (junction 24229)
          state People_IN
            state Check_People_IN
              en:
              COUNTER_IN=false;
            state Ready_IN
              en:
              IN_DEL_IN=false;
              ET_DEL_IN=0;
            state People_KID_IN
              en:
              WEIGHT=WEIGHT+30;
              KIDS=KIDS+1;
            state DELAY_IN
              state Set_tmr
                en:
                Q_DEL_IN=true;
              state Counting
                en:
                ET_DEL_IN = ET_DEL_IN + 1;
                Q_DEL_IN=false;
              state Set
                en:
                IN_DEL_IN=true;
                PT_DEL_IN=0.05;
              (junction 24312) -> Emergency.OpCl.OpCl_0.Opening0.People_IN.DELAY_IN.Set_tmr [order 1] : [ET_DEL_IN==PT_DEL_IN]
              Emergency.OpCl.OpCl_0.Opening0.People_IN.DELAY_IN.Set_tmr -> (junction 24313)
              Emergency.OpCl.OpCl_0.Opening0.People_IN.DELAY_IN.Counting -> (junction 24312)
              (junction 24312) -> (junction 24313) [order 2]
              (default) -> Emergency.OpCl.OpCl_0.Opening0.People_IN.DELAY_IN.Set
              Emergency.OpCl.OpCl_0.Opening0.People_IN.DELAY_IN.Set -> (junction 24314)
              (junction 24314) -> Emergency.OpCl.OpCl_0.Opening0.People_IN.DELAY_IN.Counting [order 1] : [ET_DEL_IN<PT_DEL_IN]
              (junction 24314) -> (junction 24313) [order 2]
            state People_WOMAN_IN
              en:
              WEIGHT=WEIGHT+55;
              WOMEN=WOMEN+1;
            state People_MAN_IN
              en:
              WEIGHT=WEIGHT+75;
              MEN=MEN+1;
            state People_FATGUY_IN
              en:
              WEIGHT=WEIGHT+100;
              FATGUYS=FATGUYS+1;
            state Re_Ready_IN
              en:
              COUNTER_IN=true;
            Emergency.OpCl.OpCl_0.Opening0.People_IN.Check_People_IN -> (junction 24257)
            (junction 24257) -> Emergency.OpCl.OpCl_0.Opening0.People_IN.People_KID_IN [order 1] : [KID_IN]
            Emergency.OpCl.OpCl_0.Opening0.People_IN.People_KID_IN -> (junction 24258)
            Emergency.OpCl.OpCl_0.Opening0.People_IN.DELAY_IN -> (junction 24259)
            (junction 24259) -> Emergency.OpCl.OpCl_0.Opening0.People_IN.Ready_IN [order 1] : [Q_DEL_IN]
            (default) -> Emergency.OpCl.OpCl_0.Opening0.People_IN.DELAY_IN
            Emergency.OpCl.OpCl_0.Opening0.People_IN.Ready_IN -> (junction 24260)
            (junction 24260) -> Emergency.OpCl.OpCl_0.Opening0.People_IN.Check_People_IN [order 1] : [COUNTER_IN]
            (junction 24257) -> (junction 24262) [order 2]
            (junction 24258) -> (junction 24261)
            (junction 24259) -> (junction 24271) [order 2]
            (junction 24260) -> (junction 24270) [order 2]
            (junction 24262) -> Emergency.OpCl.OpCl_0.Opening0.People_IN.People_WOMAN_IN [order 1] : [WOMAN_IN]
            Emergency.OpCl.OpCl_0.Opening0.People_IN.People_WOMAN_IN -> (junction 24261)
            (junction 24262) -> (junction 24263) [order 2]
            (junction 24261) -> (junction 24264)
            (junction 24263) -> Emergency.OpCl.OpCl_0.Opening0.People_IN.People_MAN_IN [order 1] : [MAN_IN]
            Emergency.OpCl.OpCl_0.Opening0.People_IN.People_MAN_IN -> (junction 24264)
            (junction 24263) -> (junction 24265) [order 2]
            (junction 24264) -> (junction 24266)
            (junction 24265) -> Emergency.OpCl.OpCl_0.Opening0.People_IN.People_FATGUY_IN [order 1] : [FATGUY_IN]
            Emergency.OpCl.OpCl_0.Opening0.People_IN.People_FATGUY_IN -> (junction 24266)
            (junction 24265) -> (junction 24267) [order 2]
            (junction 24266) -> (junction 24268)
            (junction 24267) -> (junction 24268)
            (junction 24268) -> (junction 24269)
            (junction 24270) -> (junction 24269)
            (junction 24269) -> (junction 24272)
            (junction 24271) -> (junction 24272)
            (junction 24272) -> (junction 24273)
            (junction 24273) -> Emergency.OpCl.OpCl_0.Opening0.People_IN.Re_Ready_IN [order 1] : [not(KID_IN|| WOMAN_IN || MAN_IN || FATGUY_IN)]
            (junction 24273) -> (junction 24274) [order 2]
            Emergency.OpCl.OpCl_0.Opening0.People_IN.Re_Ready_IN -> (junction 24274)
          state People_OUT
            state Ready_OUT
              en:
              IN_DEL_OUT=false;
              ET_DEL_OUT=0;
            state Check_People_OUT
              en:
              COUNTER_OUT=false;
            state People_KID_OUT
              en:
              WEIGHT=WEIGHT-30;
              KIDS=KIDS-1;
            state DELAY_OUT
              state Set_tmr
                en:
                Q_DEL_OUT=true;
              state Counting
                en:
                ET_DEL_OUT = ET_DEL_OUT + 1;
                Q_DEL_OUT=false;
              state Set
                en:
                IN_DEL_OUT=true;
                PT_DEL_OUT=0.05;
              (junction 24386) -> Emergency.OpCl.OpCl_0.Opening0.People_OUT.DELAY_OUT.Set_tmr [order 1] : [ET_DEL_OUT==PT_DEL_OUT]
              Emergency.OpCl.OpCl_0.Opening0.People_OUT.DELAY_OUT.Set_tmr -> (junction 24387)
              Emergency.OpCl.OpCl_0.Opening0.People_OUT.DELAY_OUT.Counting -> (junction 24386)
              (junction 24386) -> (junction 24387) [order 2]
              (default) -> Emergency.OpCl.OpCl_0.Opening0.People_OUT.DELAY_OUT.Set
              Emergency.OpCl.OpCl_0.Opening0.People_OUT.DELAY_OUT.Set -> (junction 24388)
              (junction 24388) -> Emergency.OpCl.OpCl_0.Opening0.People_OUT.DELAY_OUT.Counting [order 1] : [ET_DEL_OUT<PT_DEL_OUT]
              (junction 24388) -> (junction 24387) [order 2]
            state People_WOMAN_OUT
              en:
              WEIGHT=WEIGHT-55;
              WOMEN=WOMEN-1;
            state People_MAN_OUT
              en:
              WEIGHT=WEIGHT-75;
              MEN=MEN-1;
            state People_FATGUY_OUT
              en:
              WEIGHT=WEIGHT-100;
              FATGUYS=FATGUYS-1;
            state Re_Ready_OUT
              en:
              COUNTER_OUT=true;
            (default) -> Emergency.OpCl.OpCl_0.Opening0.People_OUT.DELAY_OUT
            Emergency.OpCl.OpCl_0.Opening0.People_OUT.DELAY_OUT -> (junction 24331)
            (junction 24331) -> Emergency.OpCl.OpCl_0.Opening0.People_OUT.Ready_OUT [order 1] : [Q_DEL_OUT]
            Emergency.OpCl.OpCl_0.Opening0.People_OUT.Ready_OUT -> (junction 24332)
            (junction 24332) -> Emergency.OpCl.OpCl_0.Opening0.People_OUT.Check_People_OUT [order 1] : [COUNTER_OUT]
            Emergency.OpCl.OpCl_0.Opening0.People_OUT.Check_People_OUT -> (junction 24333)
            (junction 24333) -> Emergency.OpCl.OpCl_0.Opening0.People_OUT.People_KID_OUT [order 1] : [KID_OUT && KIDS>0 ]
            Emergency.OpCl.OpCl_0.Opening0.People_OUT.People_KID_OUT -> (junction 24334)
            (junction 24331) -> (junction 24345) [order 2]
            (junction 24332) -> (junction 24343) [order 2]
            (junction 24333) -> (junction 24335) [order 2]
            (junction 24334) -> (junction 24336)
            (junction 24335) -> Emergency.OpCl.OpCl_0.Opening0.People_OUT.People_WOMAN_OUT [order 1] : [WOMAN_OUT && WOMEN>0]
            Emergency.OpCl.OpCl_0.Opening0.People_OUT.People_WOMAN_OUT -> (junction 24336)
            (junction 24335) -> (junction 24338) [order 2]
            (junction 24336) -> (junction 24337)
            (junction 24338) -> Emergency.OpCl.OpCl_0.Opening0.People_OUT.People_MAN_OUT [order 1] : [MAN_OUT && MEN>0]
            Emergency.OpCl.OpCl_0.Opening0.People_OUT.People_MAN_OUT -> (junction 24337)
            (junction 24338) -> (junction 24339) [order 2]
            (junction 24337) -> (junction 24340)
            (junction 24339) -> Emergency.OpCl.OpCl_0.Opening0.People_OUT.People_FATGUY_OUT [order 1] : [FATGUY_OUT && FATGUYS>0]
            Emergency.OpCl.OpCl_0.Opening0.People_OUT.People_FATGUY_OUT -> (junction 24340)
            (junction 24339) -> (junction 24342) [order 2]
            (junction 24340) -> (junction 24341)
            (junction 24342) -> (junction 24341)
            (junction 24341) -> (junction 24344)
            (junction 24343) -> (junction 24344)
            (junction 24344) -> (junction 24346)
            (junction 24345) -> (junction 24346)
            (junction 24346) -> (junction 24347)
            (junction 24347) -> Emergency.OpCl.OpCl_0.Opening0.People_OUT.Re_Ready_OUT [order 1] : [not(KID_OUT || WOMAN_OUT || MAN_OUT || FATGUY_OUT)]
            (junction 24347) -> (junction 24348) [order 2]
            Emergency.OpCl.OpCl_0.Opening0.People_OUT.Re_Ready_OUT -> (junction 24348)
          state BUTT_Temp1
            state Butt_temp0
              en: BUT_TEMP = 0;
              FLAG_BT=true;
              LPC0=true;
            state Butt_temp1
              en: BUT_TEMP = 1;
              FLAG_BT=true;
              LPC1=true;
            state Butt_temp2
              en: BUT_TEMP = 2;
              FLAG_BT=true;
              LPC2=true;
            state Butt_temp3
              en: BUT_TEMP = 3;
              FLAG_BT=true;
              LPC3=true;
            (default) -> (junction 24405)
            (junction 24405) -> (junction 24406) [order 1] : [not(FLAG_BT)]
            (junction 24406) -> Emergency.OpCl.OpCl_0.Opening0.BUTT_Temp1.Butt_temp0 [order 1] : [P0]
            Emergency.OpCl.OpCl_0.Opening0.BUTT_Temp1.Butt_temp0 -> (junction 24407)
            (junction 24406) -> (junction 24409) [order 2]
            (junction 24407) -> (junction 24408)
            (junction 24405) -> (junction 24416) [order 2]
            Emergency.OpCl.OpCl_0.Opening0.BUTT_Temp1.Butt_temp1 -> (junction 24408)
            (junction 24409) -> Emergency.OpCl.OpCl_0.Opening0.BUTT_Temp1.Butt_temp1 [order 1] : [P1]
            (junction 24408) -> (junction 24411)
            (junction 24409) -> (junction 24410) [order 2]
            (junction 24410) -> Emergency.OpCl.OpCl_0.Opening0.BUTT_Temp1.Butt_temp2 [order 1] : [P2]
            Emergency.OpCl.OpCl_0.Opening0.BUTT_Temp1.Butt_temp2 -> (junction 24411)
            (junction 24410) -> (junction 24412) [order 2]
            (junction 24411) -> (junction 24413)
            (junction 24412) -> Emergency.OpCl.OpCl_0.Opening0.BUTT_Temp1.Butt_temp3 [order 1] : [P3]
            Emergency.OpCl.OpCl_0.Opening0.BUTT_Temp1.Butt_temp3 -> (junction 24413)
            (junction 24413) -> (junction 24415)
            (junction 24412) -> (junction 24414) [order 2]
            (junction 24415) -> (junction 24414)
            (junction 24414) -> (junction 24417)
            (junction 24416) -> (junction 24417)
          state Opening1
            en:AP0=true;
          state Stop_Opening1
            en: AP0=false;
            FLAG_OD=true;
            IN_cl=false;
            ET_cl=0;
          (junction 24168) -> (junction 24167)
          Emergency.OpCl.OpCl_0.Opening0.Opening -> (junction 24168)
          Emergency.OpCl.OpCl_0.Opening0.Stop_Opening -> (junction 24168)
          (junction 24167) -> (junction 24171)
          (junction 24170) -> Emergency.OpCl.OpCl_0.Opening0.Opening [order 1] : [not(PA0)]
          Emergency.OpCl.OpCl_0.Opening0.Timer_open -> (junction 24169)
          (junction 24169) -> Emergency.OpCl.OpCl_0.Opening0.BUTT_Temp [order 1] : [not(FLAG==4)]
          Emergency.OpCl.OpCl_0.Opening0.BUTT_Temp -> (junction 24170)
          (junction 24170) -> Emergency.OpCl.OpCl_0.Opening0.Stop_Opening [order 2]
          (junction 24169) -> (junction 24170) [order 2]
          (junction 24172) -> Emergency.OpCl.OpCl_0.Opening0.Timer_open [order 1] : [not(OBS)]
          Emergency.OpCl.OpCl_0.Opening0.Opening1 -> (junction 24171)
          Emergency.OpCl.OpCl_0.Opening0.People_IN -> Emergency.OpCl.OpCl_0.Opening0.People_OUT
          Emergency.OpCl.OpCl_0.Opening0.People_OUT -> (junction 24172)
          (junction 24172) -> (junction 24173) [order 2]
          (junction 24173) -> Emergency.OpCl.OpCl_0.Opening0.BUTT_Temp1 [order 1] : [not(FLAG==4)]
          Emergency.OpCl.OpCl_0.Opening0.BUTT_Temp1 -> (junction 24174)
          (junction 24174) -> Emergency.OpCl.OpCl_0.Opening0.Opening1 [order 1] : [not(PA0)]
          (default) -> Emergency.OpCl.OpCl_0.Opening0.People_IN
          (junction 24173) -> (junction 24174) [order 2]
          (junction 24175) -> (junction 24171)
          (junction 24174) -> Emergency.OpCl.OpCl_0.Opening0.Stop_Opening1 [order 2]
          Emergency.OpCl.OpCl_0.Opening0.Stop_Opening1 -> (junction 24175)
        (default) -> (junction 24060)
        (junction 24060) -> (junction 24061) [order 1] : [FLAG_OD]
        (junction 24061) -> Emergency.OpCl.OpCl_0.Closing0 [order 1] : [not(SWITCH) && not(STOP) && WEIGHT<=320 && not(PS0 || P0) ]
        (junction 24060) -> Emergency.OpCl.OpCl_0.Opening0 [order 2]
        (junction 24061) -> Emergency.OpCl.OpCl_0.StopClosing [order 2]
        Emergency.OpCl.OpCl_0.Closing0 -> (junction 24062)
        Emergency.OpCl.OpCl_0.StopClosing -> (junction 24062)
        (junction 24062) -> (junction 24063)
        Emergency.OpCl.OpCl_0.Opening0 -> (junction 24063)
      state FLOOR_1
        en: CP1=false;
      state OpCl_1
        state Closing1
          state Timer_close
            state Set_tmr
              en: Q_cl=true;
            state Set
              en:PT_cl=5;
              IN_cl=true;
            state Counting
              en:ET_cl = ET_cl + 1;
              Q_cl=false;
            (junction 23720) -> Emergency.OpCl.OpCl_1.Closing1.Timer_close.Set_tmr [order 1] : [ET_cl==PT_cl]
            Emergency.OpCl.OpCl_1.Closing1.Timer_close.Set_tmr -> (junction 23721)
            (default) -> Emergency.OpCl.OpCl_1.Closing1.Timer_close.Set
            Emergency.OpCl.OpCl_1.Closing1.Timer_close.Counting -> (junction 23720)
            (junction 23720) -> (junction 23721) [order 2]
            Emergency.OpCl.OpCl_1.Closing1.Timer_close.Set -> (junction 23722)
            (junction 23722) -> Emergency.OpCl.OpCl_1.Closing1.Timer_close.Counting [order 1] : [ET_cl<PT_cl]
            (junction 23722) -> (junction 23721) [order 2]
          state BUTT_Temp
            state Butt_temp0
              en: BUT_TEMP = 0;
              FLAG_BT=true;
              LPC0=true;
            state Butt_temp1
              en: BUT_TEMP = 1;
              FLAG_BT=true;
              LPC1=true;
            state Butt_temp2
              en: BUT_TEMP = 2;
              FLAG_BT=true;
              LPC2=true;
            state Butt_temp3
              en: BUT_TEMP = 3;
              FLAG_BT=true;
              LPC3=true;
            (default) -> (junction 23735)
            (junction 23735) -> (junction 23736) [order 1] : [not(FLAG_BT)]
            (junction 23736) -> Emergency.OpCl.OpCl_1.Closing1.BUTT_Temp.Butt_temp0 [order 1] : [P0]
            Emergency.OpCl.OpCl_1.Closing1.BUTT_Temp.Butt_temp0 -> (junction 23737)
            (junction 23735) -> (junction 23744) [order 2]
            (junction 23736) -> (junction 23739) [order 2]
            (junction 23737) -> (junction 23738)
            (junction 23739) -> Emergency.OpCl.OpCl_1.Closing1.BUTT_Temp.Butt_temp1 [order 1] : [P1]
            Emergency.OpCl.OpCl_1.Closing1.BUTT_Temp.Butt_temp1 -> (junction 23738)
            (junction 23739) -> (junction 23740) [order 2]
            (junction 23738) -> (junction 23741)
            (junction 23740) -> Emergency.OpCl.OpCl_1.Closing1.BUTT_Temp.Butt_temp2 [order 1] : [P2]
            Emergency.OpCl.OpCl_1.Closing1.BUTT_Temp.Butt_temp2 -> (junction 23741)
            (junction 23740) -> (junction 23742) [order 2]
            (junction 23741) -> (junction 23743)
            (junction 23742) -> Emergency.OpCl.OpCl_1.Closing1.BUTT_Temp.Butt_temp3 [order 1] : [P3]
            Emergency.OpCl.OpCl_1.Closing1.BUTT_Temp.Butt_temp3 -> (junction 23743)
            (junction 23742) -> (junction 23745) [order 2]
            (junction 23743) -> (junction 23746)
            (junction 23744) -> (junction 23745)
            (junction 23745) -> (junction 23746)
          state Closing
            en: CP1=Q_cl;
          state Stop_Closing
            en: CP1=false;
            LPS0=false;
            LPS1=false;
            LPD1=false;
            LPS2=false;
            LPD2=false;
            LPD3=false;
            FLAG_OD=false;
            OBS=false;
            ET_cl=0;
            IN_cl=false;
          state Flag_position
            en:FLAG=2;
            FLAG_BT=false;
            BUTTON=BUT_TEMP;
          state Closing1
            en:CP1=true;
          state Flag_floor
            en: FLAG=1;
          state Stop_Closing1
            en:CP1=false;
          Emergency.OpCl.OpCl_1.Closing1.Closing -> Emergency.OpCl.OpCl_1.Closing1.BUTT_Temp
          (default) -> (junction 23687)
          (junction 23687) -> Emergency.OpCl.OpCl_1.Closing1.Timer_close [order 1] : [not(FLAG==0) && not(FLAG==4)]
          Emergency.OpCl.OpCl_1.Closing1.Timer_close -> (junction 23688)
          Emergency.OpCl.OpCl_1.Closing1.BUTT_Temp -> (junction 23689)
          (junction 23688) -> Emergency.OpCl.OpCl_1.Closing1.Closing [order 1] : [not(PC1)]
          (junction 23687) -> (junction 23691) [order 2]
          (junction 23688) -> Emergency.OpCl.OpCl_1.Closing1.Stop_Closing [order 2]
          (junction 23689) -> (junction 23693)
          Emergency.OpCl.OpCl_1.Closing1.Stop_Closing -> (junction 23690)
          (junction 23690) -> Emergency.OpCl.OpCl_1.Closing1.Flag_position [order 1] : [FLAG_BT]
          (junction 23690) -> Emergency.OpCl.OpCl_1.Closing1.Flag_floor [order 2]
          Emergency.OpCl.OpCl_1.Closing1.Flag_position -> (junction 23694)
          (junction 23691) -> Emergency.OpCl.OpCl_1.Closing1.Closing1 [order 1] : [not(PC1)]
          Emergency.OpCl.OpCl_1.Closing1.Closing1 -> (junction 23692)
          (junction 23691) -> Emergency.OpCl.OpCl_1.Closing1.Stop_Closing1 [order 2]
          (junction 23692) -> (junction 23695)
